simulink model "DLS_ex2"  (R2025b)
settings: Solver=VariableStepAuto  StartTime=0  StopTime=200000  FixedStep=0.5  MaxStep=200  MinStep=0.1  RelTol=.0001
model workspace (MATLAB code in the model file):
  | Temp_Ambient= 295.15;
  | Temp_Environment=295.15;
  | Time_Warmup = 200000;
  | 
  | %material properties: Specific heat and Density
  | Density_Copper = 8960/1000000000;
  | Density_G10 = 1800/1000000000;
  | Density_Stainless_Steel = 7930/1000000000;
  | Density_Aluminium = 2700/1000000000;
  | Density_Titanium = 4500/1000000000;
  | Density_Aluminium_Nitride = 3300/1000000000;
  | Density_Invar = 8050/1000000000;
  | 
  | SHC_Copper = 386;
  | SHC_G10 = 500;
  | SHC_Stainless_Steel = 500;
  | SHC_Aluminium = 900;
  | SHC_Titanium = 528;
  | SHC_Aluminium_Nitride = 820;
  | SHC_Phosphor_Bronze = 377;
  | SHC_Invar = 515;
  | 
  | %Radiation Coefficients
  | K_B1_LB = 2.83489E-08;
  | K_B1_RE = 1.13396E-08;
  | K_B1_UB = 5.66944E-09;
  | 
  | K_B2_LB = 5.15455E-10;
  | K_B2_RE = 2.3625E-10;
  | K_B2_UB = 9.61017E-11;
  | 
  | K_B3_LB = 5.15455E-09;
  | K_B3_RE = 2.3625E-09;
  | K_B3_UB = 9.61017E-10;
  | 
  | K_B4_LB = 5.15455E-09;
  | K_B4_RE = 2.3625E-09;
  | K_B4_UB = 9.61017E-10;
  | 
  | K_B5_LB = 5.15455E-09;
  | K_B5_RE = 2.3625E-09;
  | K_B5_UB = 9.61017E-10;
  | 
  | K_B6_LB = 5.15455E-09;
  | K_B6_RE = 2.3625E-09;
  | K_B6_UB = 9.61017E-10;
  | 
  | K_B7_LB = 5.67E-09;
  | K_B7_RE = 2.8E-09;
  | K_B7_UB = 1.11176E-09;
  | 
  | K_B8_LB = 5.67E-09;
  | K_B8_RE = 2.8E-09;
  | K_B8_UB = 1.11176E-09;
  | 
  | K_B9_LB = 2.835E-08;
  | K_B9_RE = 1.08E-08;
  | K_B9_UB = 5.15455E-09;
  | 
  | K_B10_LB = 4.78193E-09;
  | K_B10_RE = 8.95937E-10;
  | K_B10_UB = 2.20909E-09;
  | 
  | 
  | 
  | 
  | 
  | 
  | 
  | 
  | 
  | K_B13_LB = 3.54375E-09;
  | K_B13_RE = 1.73571E-09;
  | K_B13_UB = 6.85887E-10;
  | 
  | K_B14_LB = 2.98421E-09;
  | K_B14_RE = 1.45385E-09;
  | K_B14_UB = 5.72727E-10;
  | 
  | K_B15_LB = 4.05E-10;
  | K_B15_RE = 1.95517E-10;
  | K_B15_UB = 5.72727E-11;
  | 
  | K_B16_LB = 4.05E-09;
  | K_B16_RE = 1.95517E-09;
  | K_B16_UB = 5.72727E-10;
  | 
  | K_B17_LB = 2.83458E-09;
  | K_B17_RE = 1.13386E-09;
  | K_B17_UB = 5.66908E-10;
  | 
  | K_B18_LB = 2.83458E-09;
  | K_B18_RE = 1.13386E-09;
  | K_B18_UB = 5.66908E-10;
  | 
  | K_B19_LB = 2.83458E-09;
  | K_B19_RE = 1.13386E-09;
  | K_B19_UB = 5.66908E-10;
  | 
  | K_B20_LB = 5.15455E-10;
  | K_B20_RE = 2.3625E-10;
  | K_B20_UB = 9.61017E-11;
  | 
  | K_B21_LB = 9.45E-09;
  | K_B21_RE = 4.05E-09;
  | K_B21_UB = 9.61017E-10;
  | 
  | K_B22_LB = 4.78193E-09;
  | K_B22_RE = 2.20909E-09;
  | K_B22_UB = 8.95937E-10;
  | 
  | K_B23_LB = 5.15455E-09;
  | K_B23_RE = 2.3625E-09;
  | K_B23_UB = 9.61017E-10;
  | 
  | 
  | 
  | 
  | 
  | K_B25_LB = 2.98421E-09;
  | K_B25_RE = 1.45385E-09;
  | K_B25_UB = 5.72727E-10;
  | 
  | K_B1 = K_B1_RE;
  | K_B2 = K_B2_RE;
  | K_B3 = K_B3_RE;
  | K_B4 = K_B4_RE;
  | K_B5 = K_B5_RE;
  | K_B6 = K_B6_RE;
  | K_B7 = K_B7_RE;
  | K_B8 = K_B8_RE;
  | K_B9 = K_B9_RE;
  | K_B10 = K_B10_RE;
  | 
  | 
  | K_B13 = K_B13_RE;
  | K_B14 = K_B14_RE;
  | K_B15 = K_B15_RE;
  | K_B16 = K_B16_RE;
  | K_B17 = K_B17_RE;
  | K_B18 = K_B18_RE;
  | K_B19 = K_B19_RE;
  | K_B20 = K_B20_RE;
  | K_B21 = K_B21_RE;
  | K_B22 = K_B22_RE;
  | K_B23 = K_B23_RE;
  | 
  | K_B25 = K_B25_RE;
  | 
  | %Radiation Surface Area
  | Area_B1 = 100000; %measured 24400 on crude model
  | Area_B2 = 30000; %was 50900
  | Area_B3 = 450;
  | Area_B4 = 613;
  | Area_B5 = 4410;
  | Area_B6 = 1590;
  | Area_B7 = 120;
  | Area_B8 = 50;
  | Area_B9 = 140;
  | Area_B10 = 100;
  | 
  | 
  | Area_B13 = 9990;
  | Area_B14 = 7710;
  | Area_B15 = 10000; %measured 8400 on crude model for 15 and 16 combined
  | Area_B16 = 2000;
  | Area_B17 = 70015;
  | Area_B18 = 16000; %no block model in CAD, estimated value
  | Area_B19 = 320000;
  | Area_B20 = 70000;
  | Area_B21 = 4000; %no CAD, estimated value
  | Area_B22 = 4900;
  | Area_B23 = 9155;
  | 
  | Area_B25 = 4072;
  | 
  | %Akima approximation to calculate contact resistance or fixed resistance values where appropriate
  | xt=linspace(5,295,2000);
  | x_restemp=[4	10	20	30	40	50	60	70	80	90	100	110	120	130	140	150	160	170	180	190	200	210	220	230	240	250	260	273	280	293	300];
  | 
  | y_res_A1_LB=[1.852847068	0.77281194	0.49125288	0.555353451	0.801331659	1.184325573	1.60557094	1.971748902	2.248473254	2.443766462	2.578413714	2.67150152	2.736985932	2.784247759	2.819401592	2.846406384	2.867837824	2.885389229	2.900188421	2.912997223	2.924337653	2.934572526	2.943957542	2.95267538	2.960858317	2.96860341	2.975982825	2.985117154	2.989849299	2.998335893	3.002758516];
  | res_A1_LB=(akima(x_restemp,y_res_A1_LB,xt))';
  | y_res_A1_RE=[1.558179157	0.649907636	0.413126378	0.467032702	0.673891715	0.995976115	1.350228639	1.658171414	1.890886853	2.055121565	2.168355165	2.246638732	2.301708818	2.34145435	2.371017486	2.393727565	2.411750652	2.426510766	2.438956365	2.449728117	2.459265019	2.467872188	2.475764655	2.48309605	2.489977612	2.496490963	2.502696791	2.51037844	2.514358008	2.521494934	2.525214205];
  | res_A1_RE=(akima(x_restemp,y_res_A1_RE,xt))';
  | y_res_A1_UB=[1.383495056	0.577047894	0.366811672	0.414674674	0.59834317	0.884319383	1.198857421	1.472277397	1.67890361	1.824726324	1.925265549	1.994772914	2.043669212	2.078958958	2.105207835	2.125371936	2.141374494	2.154479883	2.165530233	2.175094387	2.183562128	2.191204365	2.198212025	2.204721514	2.210831598	2.216614751	2.222124857	2.228945334	2.23247876	2.238815581	2.242117892];
  | res_A1_UB=(akima(x_restemp,y_res_A1_UB,xt))';
  | 
  | y_res_A2_LB=[0.466691844	0.194654505	0.123735907	0.139881445	0.201838001	0.298305832	0.40440837	0.496640627	0.566341468	0.615531576	0.649446288	0.67289308	0.689387178	0.701291403	0.710145888	0.716947808	0.722345921	0.726766738	0.730494332	0.73372059	0.736576998	0.73915494	0.741518821	0.743714655	0.745775758	0.747726578	0.749585292	0.751886031	0.753077956	0.755215544	0.756329506];
  | res_A2_LB=(akima(x_restemp,y_res_A2_LB,xt))';
  | y_res_A2_RE=[0.422241188	0.17611439	0.111950524	0.12655826	0.182613685	0.269893315	0.365889982	0.449337462	0.512399558	0.556904491	0.587588954	0.608802526	0.623725623	0.634496015	0.642507144	0.648661206	0.653545169	0.657544919	0.660917474	0.663836444	0.666420789	0.668753191	0.670891922	0.67287861	0.674743402	0.676508414	0.678190092	0.680271694	0.681350092	0.683284083	0.684291945];
  | res_A2_RE=(akima(x_restemp,y_res_A2_RE,xt))';
  | y_res_A2_UB=[0.385689258	0.160868789	0.102259362	0.115602558	0.166805463	0.246529603	0.334216178	0.410439904	0.468042936	0.508695235	0.536723452	0.55610064	0.569731897	0.579569934	0.586887568	0.592508894	0.59697007	0.600623576	0.603704181	0.606370465	0.608731093	0.610861588	0.612815176	0.614629884	0.616333247	0.617945468	0.619481569	0.621382974	0.622368019	0.624134591	0.625055206];
  | res_A2_UB=(akima(x_restemp,y_res_A2_UB,xt))';
  | 
  | y_res_A3_LB=[0.466691844	0.194654505	0.123735907	0.139881445	0.201838001	0.298305832	0.40440837	0.496640627	0.566341468	0.615531576	0.649446288	0.67289308	0.689387178	0.701291403	0.710145888	0.716947808	0.722345921	0.726766738	0.730494332	0.73372059	0.736576998	0.73915494	0.741518821	0.743714655	0.745775758	0.747726578	0.749585292	0.751886031	0.753077956	0.755215544	0.756329506];
  | res_A3_LB=(akima(x_restemp,y_res_A3_LB,xt))';
  | y_res_A3_RE=[0.422241188	0.17611439	0.111950524	0.12655826	0.182613685	0.269893315	0.365889982	0.449337462	0.512399558	0.556904491	0.587588954	0.608802526	0.623725623	0.634496015	0.642507144	0.648661206	0.653545169	0.657544919	0.660917474	0.663836444	0.666420789	0.668753191	0.670891922	0.67287861	0.674743402	0.676508414	0.678190092	0.680271694	0.681350092	0.683284083	0.684291945];
  | res_A3_RE=(akima(x_restemp,y_res_A3_RE,xt))';
  | y_res_A3_UB=[0.385689258	0.160868789	0.102259362	0.115602558	0.166805463	0.246529603	0.334216178	0.410439904	0.468042936	0.508695235	0.536723452	0.55610064	0.569731897	0.579569934	0.586887568	0.592508894	0.59697007	0.600623576	0.603704181	0.606370465	0.608731093	0.610861588	0.612815176	0.614629884	0.616333247	0.617945468	0.619481569	0.621382974	0.622368019	0.624134591	0.625055206];
  | res_A3_UB=(akima(x_restemp,y_res_A3_UB,xt))';
  | 
  | y_res_A4_LB=[1.668225823	0.695807472	0.442303498	0.500016965	0.721485431	1.066317096	1.445588764	1.77528005	2.024431055	2.200264872	2.321495613	2.405307971	2.464267391	2.506819958	2.538470996	2.562784978	2.582080948	2.597883497	2.611208069	2.622740577	2.632951025	2.642166076	2.650615951	2.658465127	2.665832701	2.672806057	2.679450173	2.68767434	2.691934966	2.699575939	2.703557883];
  | res_A4_LB=(akima(x_restemp,y_res_A4_LB,xt))';
  | y_res_A4_RE=[1.40291919	0.585149589	0.371961671	0.420496665	0.606743849	0.896735139	1.215689261	1.492948026	1.70247525	1.8503453	1.952296086	2.022779328	2.072362125	2.108147336	2.134764744	2.155211947	2.171439179	2.184728567	2.195934063	2.205632496	2.214219123	2.221968657	2.229074704	2.235675585	2.241871455	2.247735802	2.253323269	2.260239505	2.263822541	2.27024833	2.273597005];
  | res_A4_RE=(akima(x_restemp,y_res_A4_RE,xt))';
  | y_res_A4_UB=[1.245640948	0.519549732	0.330261851	0.373355692	0.538723106	0.796204099	1.079400963	1.325576846	1.511614426	1.642907084	1.733428387	1.796009905	1.840034081	1.87180749	1.895440878	1.913595789	1.928003821	1.939803364	1.949752636	1.958363799	1.965987798	1.972868548	1.979177952	1.985038822	1.990540086	1.995746994	2.000708063	2.006848934	2.010030283	2.015735691	2.018708954];
  | res_A4_UB=(akima(x_restemp,y_res_A4_UB,xt))';
  | 
  | y_res_A5_LB=[1.101209878	0.459308357	0.291968254	0.330065398	0.476258593	0.703884871	0.954245285	1.171877272	1.336343943	1.452413323	1.532438753	1.587763994	1.626683603	1.65477291	1.675666025	1.691715889	1.704453321	1.714884717	1.723680379	1.731293084	1.738033087	1.744116019	1.749693853	1.75487516	1.759738557	1.764341728	1.768727565	1.774156407	1.776968881	1.782012752	1.784641267];
  | res_A5_LB=(akima(x_restemp,y_res_A5_LB,xt))';
  | y_res_A5_RE=[0.951197386	0.396739002	0.252194832	0.285102187	0.41138019	0.607998042	0.824253069	1.012238103	1.154300276	1.254558086	1.323682039	1.37147059	1.405088369	1.429351206	1.447398153	1.461261622	1.472263895	1.481274272	1.488871744	1.495447407	1.501269252	1.506523536	1.511341528	1.515817011	1.520017891	1.523993994	1.527782369	1.532471667	1.534901011	1.53925778	1.541528225];
  | res_A5_RE=(akima(x_restemp,y_res_A5_RE,xt))';
  | y_res_A5_UB=[0.837873198	0.34947213	0.222148729	0.251135552	0.36236899	0.535562094	0.726052831	0.891641619	1.016778724	1.105091973	1.165980605	1.208075702	1.23768831	1.25906051	1.274957372	1.287169169	1.296860648	1.304797543	1.311489863	1.317282112	1.322410351	1.327038648	1.331282632	1.335224913	1.338925306	1.342427703	1.345764737	1.349895359	1.352035275	1.355872985	1.357872932];
  | res_A5_UB=(akima(x_restemp,y_res_A5_UB,xt))';
  | 
  | y_res_A6_LB=[0.466691844	0.194654505	0.123735907	0.139881445	0.201838001	0.298305832	0.40440837	0.496640627	0.566341468	0.615531576	0.649446288	0.67289308	0.689387178	0.701291403	0.710145888	0.716947808	0.722345921	0.726766738	0.730494332	0.73372059	0.736576998	0.73915494	0.741518821	0.743714655	0.745775758	0.747726578	0.749585292	0.751886031	0.753077956	0.755215544	0.756329506];
  | res_A6_LB=(akima(x_restemp,y_res_A6_LB,xt))';
  | y_res_A6_RE=[0.422241188	0.17611439	0.111950524	0.12655826	0.182613685	0.269893315	0.365889982	0.449337462	0.512399558	0.556904491	0.587588954	0.608802526	0.623725623	0.634496015	0.642507144	0.648661206	0.653545169	0.657544919	0.660917474	0.663836444	0.666420789	0.668753191	0.670891922	0.67287861	0.674743402	0.676508414	0.678190092	0.680271694	0.681350092	0.683284083	0.684291945];
  | res_A6_RE=(akima(x_restemp,y_res_A6_RE,xt))';
  | y_res_A6_UB=[0.385689258	0.160868789	0.102259362	0.115602558	0.166805463	0.246529603	0.334216178	0.410439904	0.468042936	0.508695235	0.536723452	0.55610064	0.569731897	0.579569934	0.586887568	0.592508894	0.59697007	0.600623576	0.603704181	0.606370465	0.608731093	0.610861588	0.612815176	0.614629884	0.616333247	0.617945468	0.619481569	0.621382974	0.622368019	0.624134591	0.625055206];
  | res_A6_UB=(akima(x_restemp,y_res_A6_UB,xt))';
  | 
  | y_res_A7_LB=[0.466691844	0.194654505	0.123735907	0.139881445	0.201838001	0.298305832	0.40440837	0.496640627	0.566341468	0.615531576	0.649446288	0.67289308	0.689387178	0.701291403	0.710145888	0.716947808	0.722345921	0.726766738	0.730494332	0.73372059	0.736576998	0.73915494	0.741518821	0.743714655	0.745775758	0.747726578	0.749585292	0.751886031	0.753077956	0.755215544	0.756329506];
  | res_A7_LB=(akima(x_restemp,y_res_A7_LB,xt))';
  | y_res_A7_RE=[0.422241188	0.17611439	0.111950524	0.12655826	0.182613685	0.269893315	0.365889982	0.449337462	0.512399558	0.556904491	0.587588954	0.608802526	0.623725623	0.634496015	0.642507144	0.648661206	0.653545169	0.657544919	0.660917474	0.663836444	0.666420789	0.668753191	0.670891922	0.67287861	0.674743402	0.676508414	0.678190092	0.680271694	0.681350092	0.683284083	0.684291945];
  | res_A7_RE=(akima(x_restemp,y_res_A7_RE,xt))';
  | y_res_A7_UB=[0.385689258	0.160868789	0.102259362	0.115602558	0.166805463	0.246529603	0.334216178	0.410439904	0.468042936	0.508695235	0.536723452	0.55610064	0.569731897	0.579569934	0.586887568	0.592508894	0.59697007	0.600623576	0.603704181	0.606370465	0.608731093	0.610861588	0.612815176	0.614629884	0.616333247	0.617945468	0.619481569	0.621382974	0.622368019	0.624134591	0.625055206];
  | res_A7_UB=(akima(x_restemp,y_res_A7_UB,xt))';
  | 
  | y_res_A8_LB=[2.570275206	1.072047123	0.68146752	0.770388031	1.111609765	1.642900113	2.227252994	2.735216199	3.11908908	3.390000424	3.576783511	3.705915203	3.796755384	3.862317137	3.911082643	3.948543774	3.978273534	4.002620898	4.023150383	4.040918792	4.056650273	4.070848121	4.083867043	4.095960456	4.107311852	4.118055868	4.128292615	4.140963786	4.147528232	4.159300861	4.165435938];
  | res_A8_LB=(akima(x_restemp,y_res_A8_LB,xt))';
  | y_res_A8_RE=[2.177935172	0.908404333	0.577444811	0.652792038	0.941927931	1.392119386	1.887273636	2.317698724	2.642975273	2.872533315	3.030804871	3.140225237	3.217199105	3.272753174	3.314074863	3.345817734	3.371009391	3.391640247	3.409036006	3.424092154	3.437422301	3.449452916	3.460484563	3.470731975	3.480350635	3.48945463	3.498128787	3.508865765	3.514428181	3.524403775	3.529602362];
  | res_A8_RE=(akima(x_restemp,y_res_A8_RE,xt))';
  | y_res_A8_UB=[1.891515301	0.788940239	0.501505146	0.566943472	0.818055154	1.20904201	1.639078612	2.012898573	2.29539806	2.494766965	2.632224255	2.727254769	2.794105817	2.84235398	2.878241461	2.905809833	2.927688539	2.945606235	2.960714281	2.973790398	2.985367499	2.99581597	3.005396847	3.014296624	3.022650336	3.030557066	3.038090486	3.047415446	3.052246349	3.060910055	3.065424976];
  | res_A8_UB=(akima(x_restemp,y_res_A8_UB,xt))';
  | 
  | y_res_A9_LB=[1.302482525	0.543258029	0.34533249	0.390392805	0.56330633	0.832536797	1.128656611	1.386066089	1.580593009	1.717876865	1.812528872	1.877966134	1.923999239	1.957222544	1.98193438	2.000917743	2.015983248	2.028321232	2.038724514	2.047728624	2.055700525	2.06289526	2.069492577	2.075620893	2.081373193	2.086817704	2.092005158	2.098426252	2.101752774	2.107718533	2.110827473];
  | res_A9_LB=(akima(x_restemp,y_res_A9_LB,xt))';
  | y_res_A9_RE=[1.095341951	0.456860878	0.290412467	0.328306606	0.473720793	0.700134138	0.949160477	1.165632786	1.329223078	1.444673968	1.524272974	1.579303408	1.618015628	1.645955258	1.666737042	1.682701383	1.695370942	1.705746752	1.714495546	1.722067686	1.728771774	1.734822293	1.740370404	1.745524102	1.750361583	1.754940226	1.759302692	1.764702606	1.767500094	1.772517088	1.775131596];
  | res_A9_RE=(akima(x_restemp,y_res_A9_RE,xt))';
  | y_res_A9_UB=[0.946128819	0.394624932	0.250850982	0.283582986	0.409188103	0.604758253	0.819860939	1.006844274	1.148149452	1.247873026	1.316628644	1.364162548	1.397601191	1.42173474	1.439685522	1.453475118	1.464418764	1.473381128	1.480938116	1.48747874	1.493269562	1.498495848	1.503288167	1.507739802	1.511918297	1.515873213	1.519641402	1.524305712	1.526722111	1.531055664	1.533314011];
  | res_A9_UB=(akima(x_restemp,y_res_A9_UB,xt))';
  | 
  | y_res_A10_LB=[21.77846125	8.966644519	5.100967849	4.830535038	5.997610209	8.079798747	10.41365885	12.43492555	13.94699339	15.00095825	15.71759461	16.20529908	16.54225342	16.78052084	16.95380548	17.08380935	17.18458127	17.26531026	17.33208171	17.38897845	17.43877523	17.48338116	17.52412521	17.56194268	17.59749867	17.63127075	17.6636051	17.69475498	17.72490735	17.75420153	17.78274238];
  | res_A10_LB=(akima(x_restemp,y_res_A10_LB,xt))';
  | y_res_A10_RE=[19.70414413	8.112605106	4.615119706	4.370444611	5.426360229	7.310228083	9.421796722	11.25054532	12.61859435	13.57217298	14.2205524	14.66180485	14.96666555	15.18223888	15.33901881	15.45664029	15.54781407	15.62085392	15.68126564	15.73274318	15.777797	15.81815438	15.85501771	15.88923321	15.92140262	15.95195804	15.98121267	16.00939564	16.03667611	16.06318013	16.08900256];
  | res_A10_RE=(akima(x_restemp,y_res_A10_RE,xt))';
  | y_res_A10_UB=[17.99842591	7.410325513	4.215605081	3.992110645	4.956619375	6.677407437	8.606185031	10.27662531	11.52624717	12.39727787	12.98952937	13.39258415	13.67105413	13.86796604	14.01117409	14.11861349	14.20189467	14.26861172	14.32379381	14.37081513	14.4119688	14.44883258	14.48250478	14.51375837	14.54314299	14.57105333	14.59777549	14.62351876	14.64843765	14.67264731	14.69623439];
  | res_A10_UB=(akima(x_restemp,y_res_A10_UB,xt))';
  | 
  | res_A11_LB = 1;
  | res_A11_RE = 1;
  | res_A11_UB = 1;
  | 
  | y_res_A12_LB=[0.342532347	0.142868287	0.090816994	0.102667146	0.148140674	0.218944038	0.296818875	0.364513505	0.415671015	0.451774502	0.476666486	0.493875453	0.505981433	0.514718638	0.521217461	0.526209786	0.530171776	0.533416471	0.53615237	0.538520309	0.540616793	0.542508894	0.544243885	0.545855535	0.547368299	0.54880012	0.550164338	0.551852985	0.552727807	0.554296708	0.55511431];
  | res_A12_LB=(akima(x_restemp,y_res_A12_LB,xt))';
  | y_res_A12_RE=[0.342532347	0.142868287	0.090816994	0.102667146	0.148140674	0.218944038	0.296818875	0.364513505	0.415671015	0.451774502	0.476666486	0.493875453	0.505981433	0.514718638	0.521217461	0.526209786	0.530171776	0.533416471	0.53615237	0.538520309	0.540616793	0.542508894	0.544243885	0.545855535	0.547368299	0.54880012	0.550164338	0.551852985	0.552727807	0.554296708	0.55511431];
  | res_A12_RE=(akima(x_restemp,y_res_A12_RE,xt))';
  | y_res_A12_UB=[0.342532347	0.142868287	0.090816994	0.102667146	0.148140674	0.218944038	0.296818875	0.364513505	0.415671015	0.451774502	0.476666486	0.493875453	0.505981433	0.514718638	0.521217461	0.526209786	0.530171776	0.533416471	0.53615237	0.538520309	0.540616793	0.542508894	0.544243885	0.545855535	0.547368299	0.54880012	0.550164338	0.551852985	0.552727807	0.554296708	0.55511431];
  | res_A12_UB=(akima(x_restemp,y_res_A12_UB,xt))';
  | 
  | res_A13_LB = 7238;
  | res_A13_RE = 10000;
  | res_A13_UB = 30000;
  | 
  | y_res_A14_LB=[3232.518226	329.2505618	95.9646967	56.16367989	39.40139945	30.08010454	24.15548607	20.07156297	17.09584808	14.83878298	13.07413448	11.66127195	10.50803612	9.55148427	8.747184396	8.062910655	7.474752995	6.964623057	6.518603596	6.125826366	5.777691393	5.467312659	5.189117438	4.938552014	4.711862405	4.505928832	4.318139263	4.14629174	3.988518194	3.843224457	3.709042615];
  | res_A14_LB=(akima(x_restemp,y_res_A14_LB,xt))';
  | y_res_A14_RE=[6244.813576	636.0701578	185.3915737	108.5010775	76.11848627	58.1109315	46.66532307	38.7757037	33.02700148	28.66663912	25.25756293	22.52809243	20.30018767	18.4522513	16.89844637	15.57651664	14.44027093	13.45476486	12.59311205	11.83431646	11.16176403	10.56215184	10.0247141	9.540653605	9.102718147	8.70488071	8.342095175	8.010107643	7.705309245	7.424620246	7.165398014];
  | res_A14_RE=(akima(x_restemp,y_res_A14_RE,xt))';
  | y_res_A14_UB=[55656.95959	5668.981249	1652.30414	967.0168715	678.406723	517.9142221	415.9051296	345.588823	294.3534605	255.4916901	225.1082666	200.7818351	180.9256131	164.4558628	150.6075618	138.8258506	128.6990502	119.915718	112.2362293	105.4734565	99.47932661	94.13527734	89.34535844	85.03116475	81.12806088	77.58233099	74.34900151	71.39015952	68.67364093	66.17199759	63.86167702];
  | res_A14_UB=(akima(x_restemp,y_res_A14_UB,xt))';
  | 
  | y_res_A15_LB=[18852.89253	1919.826452	559.4350096	327.3742072	229.6417167	175.2952947	140.7570266	116.9536284	99.61203319	86.45950823	76.17664631	67.94366255	61.22351011	55.64945847	50.96263823	46.97528904	43.54809249	40.57564411	37.97683973	35.68833978	33.66002165	31.85175061	30.23104551	28.77136414	27.4508255	26.25124518	25.1573983	24.15808684	23.237513	22.39281994	21.6098224];
  | res_A15_LB=(akima(x_restemp,y_res_A15_LB,xt))';
  | y_res_A15_RE=[36421.38759	3708.86023	1080.757199	632.4452798	443.6385535	338.6481869	271.9246512	225.9395169	192.4377633	167.02876	147.1635802	131.2585039	118.2760252	107.5076672	98.45332737	90.7502765	84.12936919	78.38697743	73.36641831	68.94532783	65.0268755	61.53352611	58.40253024	55.5826117	53.03149923	50.7140628	48.60088992	46.67034743	44.891916	43.26007657	41.74742503];
  | res_A15_RE=(akima(x_restemp,y_res_A15_RE,xt))';
  | y_res_A15_UB=[86976.01305	8856.935365	2580.899808	1510.309534	1059.430054	808.7080442	649.3690541	539.5543571	459.5505696	398.872656	351.433658	313.4515763	282.448797	256.7334439	235.1112479	216.7159945	200.9049516	187.1918459	175.2025109	164.6447357	155.2872844	146.9449992	139.4680315	132.7339314	126.6417529	121.1076041	116.0612463	111.4510186	107.2040394	103.307129	99.69484483];
  | res_A15_UB=(akima(x_restemp,y_res_A15_UB,xt))';
  | 
  | res_A16_LB = 3200;
  | res_A16_RE = 15000;
  | res_A16_UB = 100000;
  | 
  | res_A17_LB = 113.53;
  | res_A17_RE = 135;
  | res_A17_UB = 166.88;
  | 
  | res_A18_LB = 113.16;
  | res_A18_RE = 134.55;
  | res_A18_UB = 166.33;
  | 
  | res_A19_LB = 2611.7;
  | res_A19_RE = 2974.3;
  | res_A19_UB = 3458;
  | 
  | y_res_A20_LB=[3.730185699	1.555839171	0.988999307	1.118047753	1.613255593	2.384305966	3.232364864	3.969561053	4.526667594	4.919835462	5.19090978	5.378315857	5.510150278	5.605298654	5.676070995	5.730437537	5.773583705	5.808918516	5.838712521	5.864499435	5.887330198	5.907935233	5.926829318	5.94438023	5.960854269	5.976446831	5.991303204	6.009692605	6.019219446	6.036304812	6.045208518];
  | res_A20_LB=(akima(x_restemp,y_res_A20_LB,xt))';
  | y_res_A20_RE=[3.136954858	1.308405972	0.831713601	0.940238801	1.356691161	2.005117381	2.71830506	3.338261103	3.806768092	4.137408428	4.365372387	4.5229743	4.633842407	4.713858842	4.77337589	4.819096238	4.855380646	4.885095978	4.910151687	4.931837574	4.951037442	4.968365551	4.984254811	4.999014511	5.012868597	5.025981393	5.03847508	5.053939918	5.061951657	5.076319848	5.083807551];
  | res_A20_RE=(akima(x_restemp,y_res_A20_RE,xt))';
  | y_res_A20_UB=[2.785277622	1.161723404	0.738471985	0.834830659	1.204595444	1.780328001	2.413561749	2.964015859	3.379999541	3.673572502	3.875979914	4.015913417	4.11435234	4.185398305	4.238243025	4.278837763	4.311054405	4.337438415	4.359685183	4.378939912	4.395987324	4.411372816	4.425480766	4.438585787	4.450886722	4.462529471	4.473622518	4.487353626	4.494467186	4.50722459	4.513872863];
  | res_A20_UB=(akima(x_restemp,y_res_A20_UB,xt))';
  | 
  | y_res_A21_LB=[5.996914074	2.501278643	1.589986221	1.797453759	2.5935854	3.833181282	5.196581594	6.381751062	7.277395496	7.909480359	8.345278875	8.646566326	8.858512797	9.01148015	9.125258843	9.212662395	9.282027269	9.338834045	9.386733025	9.428189918	9.464894289	9.498020421	9.528395908	9.556612013	9.583096859	9.608164581	9.632048752	9.661612871	9.676928904	9.704396563	9.7187108];
  | res_A21_LB=(akima(x_restemp,y_res_A21_LB,xt))';
  | y_res_A21_RE=[3.802468989	1.585988119	1.00816407	1.139713208	1.644517152	2.430508888	3.295001415	4.046482942	4.614385057	5.015171705	5.291498884	5.482536503	5.616925602	5.713917757	5.78606152	5.841481574	5.885463825	5.921483351	5.951854703	5.978141314	6.001414489	6.022418808	6.041679021	6.059570034	6.076363305	6.09225802	6.107402278	6.126148027	6.135859479	6.153275924	6.162352165];
  | res_A21_RE=(akima(x_restemp,y_res_A21_RE,xt))';
  | y_res_A21_UB=[3.349448705	1.397035944	0.888052959	1.003929536	1.448591918	2.140941812	2.902440034	3.564391213	4.064634347	4.417671892	4.661077877	4.82935557	4.947733759	5.033170419	5.096719085	5.145536479	5.184278753	5.216006969	5.242759924	5.265914789	5.286415234	5.30491713	5.321882712	5.337642217	5.352434764	5.366435807	5.379775802	5.396288211	5.404842655	5.420184132	5.428179044];
  | res_A21_UB=(akima(x_restemp,y_res_A21_UB,xt))';
  | 
  | y_res_A22_LB=[0.466691844	0.194654505	0.123735907	0.139881445	0.201838001	0.298305832	0.40440837	0.496640627	0.566341468	0.615531576	0.649446288	0.67289308	0.689387178	0.701291403	0.710145888	0.716947808	0.722345921	0.726766738	0.730494332	0.73372059	0.736576998	0.73915494	0.741518821	0.743714655	0.745775758	0.747726578	0.749585292	0.751886031	0.753077956	0.755215544	0.756329506];
  | res_A22_LB=(akima(x_restemp,y_res_A22_LB,xt))';
  | y_res_A22_RE=[0.422241188	0.17611439	0.111950524	0.12655826	0.182613685	0.269893315	0.365889982	0.449337462	0.512399558	0.556904491	0.587588954	0.608802526	0.623725623	0.634496015	0.642507144	0.648661206	0.653545169	0.657544919	0.660917474	0.663836444	0.666420789	0.668753191	0.670891922	0.67287861	0.674743402	0.676508414	0.678190092	0.680271694	0.681350092	0.683284083	0.684291945];
  | res_A22_RE=(akima(x_restemp,y_res_A22_RE,xt))';
  | y_res_A22_UB=[0.385689258	0.160868789	0.102259362	0.115602558	0.166805463	0.246529603	0.334216178	0.410439904	0.468042936	0.508695235	0.536723452	0.55610064	0.569731897	0.579569934	0.586887568	0.592508894	0.59697007	0.600623576	0.603704181	0.606370465	0.608731093	0.610861588	0.612815176	0.614629884	0.616333247	0.617945468	0.619481569	0.621382974	0.622368019	0.624134591	0.625055206];
  | res_A22_UB=(akima(x_restemp,y_res_A22_UB,xt))';
  | 
  | y_res_A23_LB=[0.466691844	0.194654505	0.123735907	0.139881445	0.201838001	0.298305832	0.40440837	0.496640627	0.566341468	0.615531576	0.649446288	0.67289308	0.689387178	0.701291403	0.710145888	0.716947808	0.722345921	0.726766738	0.730494332	0.73372059	0.736576998	0.73915494	0.741518821	0.743714655	0.745775758	0.747726578	0.749585292	0.751886031	0.753077956	0.755215544	0.756329506];
  | res_A23_LB=(akima(x_restemp,y_res_A23_LB,xt))';
  | y_res_A23_RE=[0.422241188	0.17611439	0.111950524	0.12655826	0.182613685	0.269893315	0.365889982	0.449337462	0.512399558	0.556904491	0.587588954	0.608802526	0.623725623	0.634496015	0.642507144	0.648661206	0.653545169	0.657544919	0.660917474	0.663836444	0.666420789	0.668753191	0.670891922	0.67287861	0.674743402	0.676508414	0.678190092	0.680271694	0.681350092	0.683284083	0.684291945];
  | res_A23_RE=(akima(x_restemp,y_res_A23_RE,xt))';
  | y_res_A23_UB=[0.385689258	0.160868789	0.102259362	0.115602558	0.166805463	0.246529603	0.334216178	0.410439904	0.468042936	0.508695235	0.536723452	0.55610064	0.569731897	0.579569934	0.586887568	0.592508894	0.59697007	0.600623576	0.603704181	0.606370465	0.608731093	0.610861588	0.612815176	0.614629884	0.616333247	0.617945468	0.619481569	0.621382974	0.622368019	0.624134591	0.625055206];
  | res_A23_UB=(akima(x_restemp,y_res_A23_UB,xt))';
  | 
  | y_res_A24_LB=[5.996914074	2.501278643	1.589986221	1.797453759	2.5935854	3.833181282	5.196581594	6.381751062	7.277395496	7.909480359	8.345278875	8.646566326	8.858512797	9.01148015	9.125258843	9.212662395	9.282027269	9.338834045	9.386733025	9.428189918	9.464894289	9.498020421	9.528395908	9.556612013	9.583096859	9.608164581	9.632048752	9.661612871	9.676928904	9.704396563	9.7187108];
  | res_A24_LB=(akima(x_restemp,y_res_A24_LB,xt))';
  | y_res_A24_RE=[3.802468989	1.585988119	1.00816407	1.139713208	1.644517152	2.430508888	3.295001415	4.046482942	4.614385057	5.015171705	5.291498884	5.482536503	5.616925602	5.713917757	5.78606152	5.841481574	5.885463825	5.921483351	5.951854703	5.978141314	6.001414489	6.022418808	6.041679021	6.059570034	6.076363305	6.09225802	6.107402278	6.126148027	6.135859479	6.153275924	6.162352165];
  | res_A24_RE=(akima(x_restemp,y_res_A24_RE,xt))';
  | y_res_A24_UB=[3.349448705	1.397035944	0.888052959	1.003929536	1.448591918	2.140941812	2.902440034	3.564391213	4.064634347	4.417671892	4.661077877	4.82935557	4.947733759	5.033170419	5.096719085	5.145536479	5.184278753	5.216006969	5.242759924	5.265914789	5.286415234	5.30491713	5.321882712	5.337642217	5.352434764	5.366435807	5.379775802	5.396288211	5.404842655	5.420184132	5.428179044];
  | res_A24_UB=(akima(x_restemp,y_res_A24_UB,xt))';
  | 
  | y_res_A25_LB=[3.385783654	1.412191043	0.897686592	1.014820202	1.464306299	2.164166831	2.933925815	3.603057866	4.108727656	4.465594967	4.711641429	4.881744604	5.001406965	5.087770445	5.15200849	5.201355456	5.240518008	5.272590412	5.299633585	5.323039635	5.34376247	5.362465075	5.3796147	5.395545165	5.410498182	5.424651108	5.438135816	5.454827352	5.463474596	5.478982497	5.487064139];
  | res_A25_LB=(akima(x_restemp,y_res_A25_LB,xt))';
  | y_res_A25_RE=[2.91220524	1.214664189	0.772124821	0.872874647	1.259489947	1.861459157	2.523549939	3.09908874	3.534029174	3.840980521	4.052611821	4.198922221	4.301847094	4.376130688	4.431383589	4.473828267	4.50751305	4.535099403	4.558359977	4.578492161	4.596316439	4.612403062	4.627153924	4.640856153	4.653717652	4.665890972	4.677489539	4.691846386	4.699284117	4.712622888	4.719574129];
  | res_A25_RE=(akima(x_restemp,y_res_A25_RE,xt))';
  | y_res_A25_UB=[2.557152629	1.066573771	0.677988278	0.766454804	1.105934426	1.634512263	2.215881721	2.721251514	3.103164526	3.372692728	3.558522191	3.6869946	3.777370995	3.842598021	3.891114554	3.928384427	3.957962401	3.982185459	4.002610131	4.020287823	4.035938986	4.050064347	4.063016801	4.075048471	4.086341912	4.097031075	4.107215558	4.119822035	4.126352967	4.138065491	4.144169244];
  | res_A25_UB=(akima(x_restemp,y_res_A25_UB,xt))';
  | 
  | y_res_A26_LB=[0.466691844	0.194654505	0.123735907	0.139881445	0.201838001	0.298305832	0.40440837	0.496640627	0.566341468	0.615531576	0.649446288	0.67289308	0.689387178	0.701291403	0.710145888	0.716947808	0.722345921	0.726766738	0.730494332	0.73372059	0.736576998	0.73915494	0.741518821	0.743714655	0.745775758	0.747726578	0.749585292	0.751886031	0.753077956	0.755215544	0.756329506];
  | res_A26_LB=(akima(x_restemp,y_res_A26_LB,xt))';
  | y_res_A26_RE=[0.422241188	0.17611439	0.111950524	0.12655826	0.182613685	0.269893315	0.365889982	0.449337462	0.512399558	0.556904491	0.587588954	0.608802526	0.623725623	0.634496015	0.642507144	0.648661206	0.653545169	0.657544919	0.660917474	0.663836444	0.666420789	0.668753191	0.670891922	0.67287861	0.674743402	0.676508414	0.678190092	0.680271694	0.681350092	0.683284083	0.684291945];
  | res_A26_RE=(akima(x_restemp,y_res_A26_RE,xt))';
  | y_res_A26_UB=[0.385689258	0.160868789	0.102259362	0.115602558	0.166805463	0.246529603	0.334216178	0.410439904	0.468042936	0.508695235	0.536723452	0.55610064	0.569731897	0.579569934	0.586887568	0.592508894	0.59697007	0.600623576	0.603704181	0.606370465	0.608731093	0.610861588	0.612815176	0.614629884	0.616333247	0.617945468	0.619481569	0.621382974	0.622368019	0.624134591	0.625055206];
  | res_A26_UB=(akima(x_restemp,y_res_A26_UB,xt))';
  | 
  | y_res_A27_LB=[0.466691844	0.194654505	0.123735907	0.139881445	0.201838001	0.298305832	0.40440837	0.496640627	0.566341468	0.615531576	0.649446288	0.67289308	0.689387178	0.701291403	0.710145888	0.716947808	0.722345921	0.726766738	0.730494332	0.73372059	0.736576998	0.73915494	0.741518821	0.743714655	0.745775758	0.747726578	0.749585292	0.751886031	0.753077956	0.755215544	0.756329506];
  | res_A27_LB=(akima(x_restemp,y_res_A27_LB,xt))';
  | y_res_A27_RE=[0.422241188	0.17611439	0.111950524	0.12655826	0.182613685	0.269893315	0.365889982	0.449337462	0.512399558	0.556904491	0.587588954	0.608802526	0.623725623	0.634496015	0.642507144	0.648661206	0.653545169	0.657544919	0.660917474	0.663836444	0.666420789	0.668753191	0.670891922	0.67287861	0.674743402	0.676508414	0.678190092	0.680271694	0.681350092	0.683284083	0.684291945];
  | res_A27_RE=(akima(x_restemp,y_res_A27_RE,xt))';
  | y_res_A27_UB=[0.385689258	0.160868789	0.102259362	0.115602558	0.166805463	0.246529603	0.334216178	0.410439904	0.468042936	0.508695235	0.536723452	0.55610064	0.569731897	0.579569934	0.586887568	0.592508894	0.59697007	0.600623576	0.603704181	0.606370465	0.608731093	0.610861588	0.612815176	0.614629884	0.616333247	0.617945468	0.619481569	0.621382974	0.622368019	0.624134591	0.625055206];
  | res_A27_UB=(akima(x_restemp,y_res_A27_UB,xt))';
  | 
  | y_res_A28_LB=[3.385783654	1.412191043	0.897686592	1.014820202	1.464306299	2.164166831	2.933925815	3.603057866	4.108727656	4.465594967	4.711641429	4.881744604	5.001406965	5.087770445	5.15200849	5.201355456	5.240518008	5.272590412	5.299633585	5.323039635	5.34376247	5.362465075	5.3796147	5.395545165	5.410498182	5.424651108	5.438135816	5.454827352	5.463474596	5.478982497	5.487064139];
  | res_A28_LB=(akima(x_restemp,y_res_A28_LB,xt))';
  | y_res_A28_RE=[2.91220524	1.214664189	0.772124821	0.872874647	1.259489947	1.861459157	2.523549939	3.09908874	3.534029174	3.840980521	4.052611821	4.198922221	4.301847094	4.376130688	4.431383589	4.473828267	4.50751305	4.535099403	4.558359977	4.578492161	4.596316439	4.612403062	4.627153924	4.640856153	4.653717652	4.665890972	4.677489539	4.691846386	4.699284117	4.712622888	4.719574129];
  | res_A28_RE=(akima(x_restemp,y_res_A28_RE,xt))';
  | y_res_A28_UB=[2.557152629	1.066573771	0.677988278	0.766454804	1.105934426	1.634512263	2.215881721	2.721251514	3.103164526	3.372692728	3.558522191	3.6869946	3.777370995	3.842598021	3.891114554	3.928384427	3.957962401	3.982185459	4.002610131	4.020287823	4.035938986	4.050064347	4.063016801	4.075048471	4.086341912	4.097031075	4.107215558	4.119822035	4.126352967	4.138065491	4.144169244];
  | res_A28_UB=(akima(x_restemp,y_res_A28_UB,xt))';
  | 
  | res_A31_LB = 113.53;
  | res_A31_RE = 135;
  | res_A31_UB = 166.88;
  | 
  | res_A32_LB = 113.53;
  | res_A32_RE = 135;
  | res_A32_UB = 166.88;
  | 
  | res_A33_LB = 113.53;
  | res_A33_RE = 135;
  | res_A33_UB = 166.88;
  | 
  | res_A34_LB = 106.89;
  | res_A34_RE = 127.1;
  | res_A34_UB = 157.12;
  | 
  | res_A36_LB = 100;
  | res_A36_RE = 100;
  | res_A36_UB = 100;
  | 
  | y_res_A37_LB=[559.0264465	277.2362191	143.0749777	104.5075798	87.00904569	78.13471948	71.71197015	67.96291148	65.29305409	62.842993	60.67239457	58.91033361	57.3420793	55.60751686	53.98751593	52.67332244	51.36613692	50.09621037	48.99723247	48.01630621	46.85892867	45.6703913	44.78832759	44.04526831	43.31563014	42.56138686	41.81566865	40.7882804	40.20917218	39.33052889	38.95803316];
  | res_A37_LB=(akima(x_restemp,y_res_A37_LB,xt))';
  | y_res_A37_RE=[647.1900089	320.958896	165.6392048	120.9893771	100.7311647	90.45727643	83.02160102	78.68128165	75.59036344	72.75390539	70.24098382	68.20102979	66.38544749	64.37732876	62.50183893	60.98038516	59.46704457	57.99683904	56.72454231	55.58891505	54.24900852	52.87302799	51.8518548	50.9916083	50.14689955	49.27370523	48.41038047	47.22096373	46.55052488	45.53331153	45.10206983];
  | res_A37_RE=(akima(x_restemp,y_res_A37_RE,xt))';
  | y_res_A37_UB=[769.5803815	381.6555667	196.963304	143.8697286	119.7804773	107.5636897	98.72185062	93.56073165	89.8852886	86.51242679	83.52428557	81.09855499	78.93962716	76.55175226	74.32158777	72.51241124	70.71288218	68.96464546	67.45174417	66.10135796	64.50806116	62.87186837	61.6575807	60.63465262	59.63020065	58.59187618	57.56528771	56.15093988	55.35371406	54.14413507	53.63134107];
  | res_A37_UB=(akima(x_restemp,y_res_A37_UB,xt))';
  | 
  | y_res_A38_LB=[2345.090752	1130.561947	581.6666576	422.6544105	349.8576636	312.0465495	284.8066406	268.4066012	256.6420417	246.1348008	236.9762773	229.5566373	223.0182223	215.9827861	209.4645901	204.153488	198.9254688	193.8820407	189.5114151	185.6109261	181.0822346	176.460892	172.997342	170.0672492	167.2022427	164.2593883	161.3602236	157.4235406	155.1660155	151.8003204	150.3265927];
  | res_A38_LB=(akima(x_restemp,y_res_A38_LB,xt))';
  | y_res_A38_RE=[2714.932924	1308.861864	673.4007875	489.3108607	405.0334038	361.2591326	329.723242	310.736767	297.1168293	284.9525007	274.3495947	265.7598099	258.1902273	250.0452388	242.4990638	236.3503526	230.2978272	224.4590044	219.3990914	214.8834598	209.6405524	204.290382	200.2805986	196.8884035	193.5715593	190.1645899	186.8082006	182.2506669	179.6371095	175.7406136	174.0344656];
  | res_A38_RE=(akima(x_restemp,y_res_A38_RE,xt))';
  | y_res_A38_UB=[3228.355021	1556.381277	800.7478913	581.8446417	481.6294397	429.5769979	392.0773418	369.5003266	353.3047168	338.839987	326.231961	316.0177584	307.0166889	297.3313982	288.358163	281.0466664	273.8495453	266.9065404	260.8897451	255.5201605	249.2857647	242.9238213	238.1557461	234.1220516	230.1779576	226.1266948	222.1355773	216.7161665	213.6083582	208.9749944	206.946196];
  | res_A38_UB=(akima(x_restemp,y_res_A38_UB,xt))';
  | 
  | res_A1 = res_A1_RE;
  | res_A2 = res_A2_RE;
  | res_A3 = res_A3_RE;
  | res_A4 = res_A4_RE;
  | res_A5 = res_A5_RE;
  | res_A6 = res_A6_RE;
  | res_A7 = res_A7_RE;
  | res_A8 = res_A8_RE;
  | res_A9 = res_A9_RE;
  | res_A10 = res_A10_RE;
  | res_A11 = res_A11_RE;
  | res_A12 = res_A12_RE;
  | res_A13 = res_A13_RE;
  | res_A14 = res_A14_RE;
  | res_A15 = res_A15_RE;
  | res_A16 = res_A16_RE;
  | res_A17 = res_A17_RE;
  | res_A18 = res_A18_RE;
  | res_A19 = res_A19_RE;
  | res_A20 = res_A20_RE;
  | res_A21 = res_A21_RE;
  | res_A22 = res_A22_RE;
  | res_A23 = res_A23_RE;
  | res_A24 = res_A24_RE;
  | res_A25 = res_A25_RE;
  | res_A26 = res_A26_RE;
  | res_A27 = res_A27_RE;
  | res_A28 = res_A28_RE;
  | 
  | res_A31 = res_A31_RE;
  | res_A32 = res_A32_RE;
  | res_A33 = res_A33_RE;
  | res_A34 = res_A34_RE;
  | 
  | res_A36 = res_A36_RE;
  | res_A37 = res_A37_RE;
  | res_A38 = res_A38_RE;
  | 
  | %Component Geometry
  | Length_1_2_1 = 35;
  | Length_1_2_2 = 280;
  | Length_1_2_3 = 25.4;
  | Length_1_3 = 442;
  | Length_1_4_1 = 25.4;
  | Length_1_4_2_3D = 370;
  | Length_1_4_2_2D = 100;
  | Length_1_4_2 = Length_1_4_2_2D;
  | Length_1_4_3 = 25.4;
  | Length_1_5_1 = 10.5;
  | Length_1_5_2 = 14;
  | Length_1_6_1 = 2.5;
  | Length_1_6_2 = 4.55;
  | Length_1_6_3 = 2.5;
  | Length_1_7 = 2;
  | Length_1_8 = 0.25;
  | 
  | Length_2_2 = 1.5;
  | Length_2_3_1 = 25;
  | Length_2_3_2 = 285;
  | Length_2_3_3 = 25;
  | Length_2_4_1 = 270;
  | Length_2_4_2 = 390;
  | Length_2_4_3 = 150;
  | Length_2_5_1 = 25;
  | Length_2_5_2 = 50;
  | Length_2_5_3 = 25;
  | Length_2_6 = 25;
  | 
  | Length_3_1 = 10;
  | 
  | %Length_4_1 = 5;
  | Length_4_2 = 5;
  | Length_4_3 = 5;
  | Length_4_4 = 25;
  | Length_4_7_1 = 5.5; %outer ring
  | Length_4_7_2 = 12.3; %outer arm
  | Length_4_7_3 = 36.3; %inner ring arm
  | Length_4_7_4 = 12; %flexure
  | Length_4_7_5 = 1.1; %inner arm
  | Length_4_7_6 = 5.8; %connector
  | 
  | Length_7_1_1 = 170;
  | Length_7_1_2 = 50;
  | Length_7_1_3_1 = 1;
  | Length_7_1_3_2 = 1;
  | Length_7_3 = 12;
  | Length_7_4_1 = 12;
  | Length_7_4_2 = 12;
  | 
  | Area_1_2_1 = 711.2;
  | Area_1_2_2 = 232.6;
  | Area_1_2_3 = 711.2;
  | Area_1_3 = 560;
  | Area_1_4_1 = 160;
  | Area_1_4_2 = 12.9;
  | Area_1_4_3 = 160;
  | Area_1_5_1 = 43.5;
  | Area_1_5_2 = 300;
  | Area_1_6_1 = 291.2;
  | Area_1_6_2 = 1040;
  | Area_1_6_3 = 1040;
  | Area_1_7 = 40;
  | Area_1_8 = 0.62;
  | 
  | Area_2_2 = 39100;
  | Area_2_3_1 = 230;
  | Area_2_3_2 = 230;
  | Area_2_3_3 = 230;
  | Area_2_4_1 = 1230;
  | Area_2_4_2 = 220;
  | Area_2_4_3 = 1000;
  | Area_2_5_1 = 161;
  | Area_2_5_2 = 25;
  | Area_2_5_3 = 161;
  | Area_2_6 = 150;
  | 
  | Area_3_1 = 50;
  | 
  | %Area_4_1 = 1*5;
  | Area_4_2 = 6*5;
  | Area_4_3 = 6*5;
  | Area_4_4 = 6*4;
  | Area_4_7_1 = 650.3;
  | Area_4_7_2 = 6;
  | Area_4_7_3 = 6;
  | Area_4_7_4 = 0.8;
  | Area_4_7_5 = 8;
  | Area_4_7_6 = 30;
  | 
  | 
  | Area_7_1_1 = 0.0544;
  | Area_7_1_2 = 0.0544;
  | Area_7_1_3_1 = 0.0544;
  | Area_7_1_3_2 = 20;
  | Area_7_3 = 33.6;
  | Area_7_4_1 = 33.6;
  | Area_7_4_2 = 33.6;
  | 
  | Mass_1_2_1 = Length_1_2_1*Area_1_2_1*Density_Copper;
  | Mass_1_2_2 = Length_1_2_2*Area_1_2_2*Density_Copper;
  | Mass_1_2_3 = Length_1_2_3*Area_1_2_3*Density_Copper;
  | Mass_1_3 = Length_1_3*Area_1_3*Density_Copper;
  | Mass_1_4_1 = Length_1_4_1*Area_1_4_1*Density_Copper;
  | Mass_1_4_2 = Length_1_4_2*Area_1_4_2*Density_Copper;
  | Mass_1_4_3 = Length_1_4_3*Area_1_4_3*Density_Copper;
  | Mass_1_5_1 = Length_1_5_1*Area_1_5_1*Density_Copper;
  | Mass_1_5_2 = Length_1_5_2*Area_1_5_2*Density_Copper;
  | Mass_1_6_1 = Length_1_6_1*Area_1_6_1*Density_Copper;
  | Mass_1_6_2 = Length_1_6_2*Area_1_6_2*Density_Copper;
  | Mass_1_6_3 = Length_1_6_3*Area_1_6_3*Density_Copper;
  | Mass_1_7 = Length_1_7*Area_1_7*Density_Copper;
  | Mass_1_8 = Length_1_8*Area_1_8*Density_Copper;
  | 
  | Mass_2_2 = Length_2_2*Area_2_2*Density_Copper;
  | Mass_2_3_1 = Length_2_3_1*Area_2_3_1*Density_Copper;
  | Mass_2_3_2 = Length_2_3_2*Area_2_3_2*Density_Copper;
  | Mass_2_3_3 = Length_2_3_3*Area_2_3_3*Density_Copper;
  | Mass_2_4_1 = Length_2_4_1*Area_2_4_1*Density_Copper;
  | Mass_2_4_2 = Length_2_4_2*Area_2_4_2*Density_Copper;
  | Mass_2_4_3 = Length_2_4_3*Area_2_4_3*Density_Copper;
  | Mass_2_5_1 = Length_2_5_1*Area_2_5_1*Density_Copper;
  | Mass_2_5_2 = Length_2_5_2*Area_2_5_2*Density_Copper;
  | Mass_2_5_3 = Length_2_5_3*Area_2_5_3*Density_Copper;
  | Mass_2_6 = Length_2_6*Area_2_6*Density_Copper;
  | 
  | Mass_3_1 = Length_3_1*Area_3_1*Density_Aluminium;
  | 
  | %Mass_4_1 = Length_4_1*Area_4_1*Density_G10;
  | Mass_4_2 = Length_4_2*Area_4_2*Density_G10;
  | Mass_4_3 = Length_4_3*Area_4_3*Density_G10;
  | Mass_4_4 = Length_4_4*Area_4_4*Density_G10;
  | Mass_4_7_1 = Length_4_7_1*Area_4_7_1*Density_Titanium;
  | Mass_4_7_2 = Length_4_7_2*Area_4_7_2*Density_Titanium;
  | Mass_4_7_3 = Length_4_7_3*Area_4_7_3*Density_Titanium;
  | Mass_4_7_4 = Length_4_7_4*Area_4_7_4*Density_Titanium;
  | Mass_4_7_5 = Length_4_7_5*Area_4_7_5*Density_Titanium;
  | Mass_4_7_6 = Length_4_7_6*Area_4_7_6*Density_Titanium;
  | 
  | Mass_4_7 = Mass_4_7_1+(6*Mass_4_7_2)+(3*Mass_4_7_3)+(6*Mass_4_7_4)+(3*Mass_4_7_5)+(3*Mass_4_7_6);
  | 
  | %no phosphor bronze or Polyimide in code (being lazy)
  | Mass_7_1_1 = Length_7_1_1*Area_7_1_1*Density_G10;
  | Mass_7_1_2 = Length_7_1_2*Area_7_1_2*Density_G10;
  | Mass_7_1_3 = Length_7_1_3_2*Area_7_1_3_2*Density_G10;
  | Mass_7_3 = Length_7_3*Area_7_3*Density_Copper;
  | Mass_7_4 = Length_7_4_2*Area_7_4_2*Density_Copper;
  | 
  | %Material Conductivities - Akima
  | x_Copper=[4	10	20	30	40	50	60	70	80	90	100	110	120	130	140	150	160	170	180	190	200	210	220	230	240	250	260	270	280	290	300];
  | y_Copper=[1300	1539.915576	2422.510265	2142.896819	1485.109355	1004.846277	741.2099419	603.5581619	529.2769842	486.9798983	461.5493381	445.4667663	434.8086444	427.4278894	422.0984859	418.093899	414.9694705	412.4452713	410.3406298	408.5363123	406.9520296	405.5327079	404.2399139	403.0463867	401.9324857	400.8838429	399.8897888	398.9422797	398.0351596	397.1636446	396.323959];
  | Cond_Copper=(akima(x_Copper,y_Copper,xt))';
  | x_Stainless_Steel=[4	10	20	30	40	50	60	70	80	90	100	110	120	130	140	150	160	170	180	190	200	210	220	230	240	250	260	270	280	290	300];
  | y_Stainless_Steel=[0.272396189	0.903857571	2.168622406	3.468572587	4.670281	5.730166936	6.646641427	7.434751536	8.114319471	8.704844967	9.223590217	9.685093439	10.10128078	10.48179376	10.83436242	11.16515436	11.4790756	11.78001966	12.07106923	12.35465738	12.63269588	12.90667672	13.17775271	13.44680137	13.7144757	13.98124475	14.24742608	14.51321188	14.77869006	15.04386145	15.30865382];
  | Cond_Stainless_Steel=(akima(x_Stainless_Steel,y_Stainless_Steel,xt))';
  | x_G10=[4	10	20	30	40	50	60	70	80	90	100	110	120	130	140	150	160	170	180	190	200	210	220	230	240	250	260	273	280	290	300];
  | y_G10=[0.072322856	0.112201845	0.15642187	0.191111597	0.217459505	0.238163639	0.255310109	0.270284605	0.283977369	0.296959296	0.309599321	0.32213809	0.334733685	0.347490177	0.36047569	0.373733984	0.387292023	0.401164973	0.415359572	0.429876425	0.444711587	0.459857685	0.475304701	0.491040551	0.507051498	0.523322473	0.539837305	0.561642965	0.573529445	0.590670406	0.607982755];
  | Cond_G10=(akima(x_G10,y_G10,xt))';
  | %x_Titanium=[2.0515	2.2546	2.4392	2.6388	2.8548	3.3943	4.3661	5.5284	6.7832	8.3229	10.212	13.989	17.994	23.512	33.766	52.459	78.976	117.04	181.84	241.37	310.48];
  | %y_Titanium=[0.12232	0.13924	0.1551	0.16909	0.18836	0.23375	0.31623	0.42781	0.51955	0.65879	0.81752	1.1301	1.4643	1.8973	2.5119	3.3982	4.403	5.7049	7.5531	9.1728	10.902];
  | %Cond_Titanium=(akima(x_Titanium,y_Titanium,xt))';
  | x_Ti6Al4V = [3.386124876 20.75387993 27.4220298	36.75105129	43.85874494	52.73850131	64.27774056	76.69884488	88.67346161	105.0768464	120.1449347	132.5535402	150.7206551	168.4454488	181.2949868	194.5896236	208.7702918	225.6104428	238.0176595	250.4276537	268.1524474	283.662857	294.7403323 295];
  | y_Ti6Al4V = [0.205026155 1.358500785 1.684540973	2.078506201	2.377376374	2.703416562	3.083796782	3.437006986	3.749462166	4.116257378	4.401542543	4.632487677	4.944942857	5.257398038	5.474758163	5.719288305	5.977403454	6.289858634	6.50721876	6.751748901	7.064204082	7.349489246	7.539679356 7.543];
  | Cond_Titanium=(akima(x_Ti6Al4V,y_Ti6Al4V,xt))';
  | x_Aluminium=[4	10	20	30	40	50	60	70	80	90	100	110	120	130	140	150	160	170	180	190	200	210	220	230	240	250	260	270	280	290	300];
  | y_Aluminium=[5.347423899	14.20430536	28.42754763	41.098463	52.23304247	62.04805557	70.75945479	78.548489	85.56117329	91.91421797	97.70122297	102.9978192	107.8656678	112.3555088	116.5094768	120.3628668	123.9454888	127.2827167	130.3963069	133.3050423	136.0252443	138.5711815	140.9554008	143.1889946	145.2818209	147.2426834	149.0794814	150.799334	152.4086848	153.9133894	155.3187898];
  | Cond_Aluminium=(akima(x_Aluminium,y_Aluminium,xt))';
  | x_Aluminium_Nitride=[4.510967205	5.519278711	6.893424895	8.194672663	11.02220728	15.96576668	18.06467613	20.95070596	24.90549764	30.3472866	35.19559795	39.98681034	49.94240884	59.61479584	70.28693352	79.85516497	99.32709193	124.5685636	149.9232744	175.3127763	200	225.3628799	247.746023	273.4758701	289.7018044 296];
  | y_Aluminium_Nitride=[0.146286823	0.259224634	0.485333553	0.77895911	1.720179013	4.383096438	5.835067139	8.207464275	11.80186514	17.15921944	22.34846936	28.47245162	39.61964949	50.48375339	60.88500046	68.73555234	83.82675	93.62855647	100.0662615	100.1129163	101.2590518	101.2950791	99.12069462	96.99417489	95.95043888 95];
  | Cond_Aluminium_Nitride=(akima(x_Aluminium_Nitride,y_Aluminium_Nitride,xt))';
  | x_Phosphor_Bronze = [4 10	20	30	40	50	60	70	80	90	100	110	120	130	140	150	160	170	180	190	200	210	220	230	240	250	260	270	280	290 300];
  | y_Phosphor_Bronze = [1 4.393242753	9.479425007	13.56115329	16.94081133	19.93208133	22.70978973	25.3722085	27.97919185	30.57036336	33.17382604	35.81054343	38.49667497	41.24489339	44.06516619	46.96523874	49.95094198	53.02639195	56.19412002	59.45515736	62.80908905	66.25408831	69.78693823	73.40304697	77.09646061	80.85987755	84.68466721	88.5608958	92.47736095	96.42163718	98.3801333];
  | Cond_Phosphor_Bronze=(akima(x_Phosphor_Bronze,y_Phosphor_Bronze,xt))';
  | x_Invar = [4	10	20	30	40	50	60	70	80	90	100	110	120	130	140	150	160	170	180	190	200	210	220	230	240	250	260	270	280	290	300];
  | y_Invar = [0.241863429	0.733851185	1.652068813	2.570059877	3.43704896	4.247347833	5.005323106	5.716516689	6.385642999	7.016349158	7.611390432	8.172859892	8.702383399	9.201266957	9.670602925	10.11134476	10.52435878	10.9104594	11.27043275	11.60505191	11.91508648	12.20130795	12.46449231	12.70542074	12.92487899	13.12365589	13.3025415	13.46232477	13.60379132	13.72772106	13.83488599];
  | Cond_Invar =(akima(x_Invar,y_Invar,xt))';
  | x_ti_15_3_3_3 = [1.425338153	1.621392126	1.820795595	2.031588851	2.23775962	2.545561431	2.877101768	3.33672869	3.820230365	4.345699594	4.84880064	5.480320658	6.15430626	6.778860806	7.661756725	8.54875725	9.295731738	10.30527775	11.57265046	12.74707226	14.13144482	15.66616465	17.36755992	19.25373213	21.07143098	22.91261337	25.40099601	27.97875325	30.81810781	33.94560725	37.15033091	40.65760489	44.78364134	49.01155791	55.03914031	61.01656589	68.08044535	77.94549955	87.53146134	96.41437516	106.1987495	119.2593773	130.5183701	141.9228222	151.3691295	160.4072083	171.0838265	181.2990475	190.8901776	211.6214577	219.9635632	231.6001338	242.2860213	251.8369222	297.7697642];
  | y_ti_15_3_3_3 = [0.028183829	0.036192676	0.045927094	0.055568361	0.062596741	0.070514083	0.077563103	0.086338977	0.094969949	0.108263673	0.119086373	0.130990976	0.145811945	0.1603882	0.180674371	0.201116766	0.216014428	0.240455371	0.267661685	0.294418786	0.323850691	0.360492764	0.396529828	0.436169378	0.474091391	0.515310469	0.573615251	0.638516925	0.702346988	0.772557894	0.83972664	0.934737476	1.04049831	1.144512894	1.289272821	1.45234223	1.616667433	1.842965653	2.027199786	2.203451259	2.366671228	2.66601181	2.897803719	3.075608373	3.264322838	3.423597958	3.633664514	3.81096081	3.949587358	4.242151817	4.556387898	4.722129913	4.952535374	5.011872336	5.992198712];
  | Cond_ti_15_3_3_3 =(akima(x_ti_15_3_3_3,y_ti_15_3_3_3,xt))';
  | x_Inconel_718 = [1.993355482	5.980066445	11.96013289	16.61129568	21.59468439	27.90697674	35.54817276	45.18272425	56.47840532	70.09966777	82.72425249	103.3222591	119.6013289	137.8737542	155.8139535	178.7375415	209.3023256	235.8803987	257.807309	275.4152824	293.3554817	300];
  | y_Inconel_718 = [0.576923077	0.892857143	1.826923077	2.513736264	3.186813187	3.846153846	4.450549451	5.068681319	5.645604396	6.195054945	6.634615385	7.225274725	7.596153846	7.93956044	8.228021978	8.516483516	8.818681319	9.07967033	9.299450549	9.491758242	9.725274725	9.848901099];
  | Cond_Inconel_718 =(akima(x_Inconel_718,y_Inconel_718,xt))';
  | x_Hastelloy_X = [4 6.264716558	6.644418163	7.122895706	7.474157486	7.96974	8.407624459	8.917265994	9.457611695	10.1931282	11.04477788	12.09640607	13.10699009	14.50949219	15.89111865	17.4043067	19.16396477	21.32853298	23.6112449	26.27848232	28.62778213	31.69191561	35.27292132	38.42658056	42.31309642	46.84357442	52.69854316	58.6539576	65.28325575	73.83893523	84.41542344	94.96838333	107.9913683	122.8001913	137.4127464	153.7651381	172.0623536	191.5095093	214.2952513	241.0831752	264.0536959	284.6023373	301.8659978];
  | y_Hastelloy_X = [0.7 0.846137913	0.900733102	0.973957115	1.03141131	1.097960859	1.168804371	1.237752699	1.331418781	1.439654868	1.564822259	1.709757645	1.86811709	2.051807187	2.230196716	2.4240959	2.634853191	2.893935687	3.129194704	3.401255144	3.62071366	3.894708671	4.146006192	4.390581075	4.649583548	4.872819029	5.160268949	5.436275753	5.667673067	5.908919904	6.160435512	6.422656985	6.696040023	6.981059723	7.316233877	7.627652383	7.993870698	8.334133095	8.825767583	9.249509722	9.64321891	10.05368649	10.31905456];
  | Cond_Hastelloy_X = (akima(x_Hastelloy_X,y_Hastelloy_X,xt))';
  | 
  | %Cond_4_7 = Cond_Hastelloy_X;
  | Cond_4_7 = Cond_Titanium;
  | 
  | x_heater=[4,65,296];
  | y_heater=[48,49,0];
  | WATTAGE_HEATER=(akima(x_heater,y_heater,xt))';
  | 
  | %Cryocooler algebraic loop parameters
  | TEMP_COLD_HEAD=linspace(2.91,299,2000);
  | x_COLD_HEAD=[2.907692308	4.371428571	5.854945055	6.389010989	7.476923077	15.52747253 18.49148418	20.1946472	21.89781022	23.84428224	25.79075426	27.73722628	29.9270073	32.36009732	34.54987835	37.46958637	40.1459854	43.55231144	46.71532847	49.8783455	52.55474453	55.71776156	58.63746959	61.55717762	64.72019465	67.63990268	70.80291971	74.20924574	77.85888078	81.99513382	85.88807786	89.5377129	93.43065693	97.08029197	100.973236	104.86618	109.7323601	114.5985401	119.2214112	124.8175182	130.4136253	136.4963504	142.8223844	149.3917275	156.9343066	164.7201946	172.5060827	181.0218978	188.8077859	197.56691	206.5693431	214.3552311	221.6545012	230.1703163	238.6861314	248.1751825	257.4209246	265.6934307	273.4793187	281.9951338	292.2141119	299.756691];
  | y_COLD_HEAD=[0	1	1.25	1.5	2	5 5.483870968	6.182795699	6.989247312	7.688172043	8.440860215	9.139784946	9.838709677	10.43010753	11.02150538	11.66666667	12.25806452	12.95698925	13.5483871	14.24731183	14.78494624	15.43010753	16.02150538	16.61290323	17.20430108	17.79569892	18.38709677	18.97849462	19.62365591	20.37634409	21.02150538	21.82795699	22.74193548	23.60215054	24.40860215	25.21505376	26.07526882	26.88172043	27.58064516	28.33333333	28.97849462	29.51612903	29.94623656	30.37634409	30.80645161	31.1827957	31.50537634	31.82795699	32.09677419	32.3655914	32.58064516	32.79569892	33.01075269	33.17204301	33.44086022	33.70967742	33.92473118	34.13978495	34.30107527	34.51612903	34.83870968	35.05376344];
  | WATTAGE_COLD_HEAD=(akima(x_COLD_HEAD,y_COLD_HEAD,TEMP_COLD_HEAD))';
libraries: fl_lib x606, nesl_utility x187, slpidlib x8, simulink x2
(part 1 of 17)
settings Model: Creator=fco17919  LastModifiedBy=lyu87474
settings SolverCC: InitialStep=0.5  MaxConsecutiveMinStep=5  ZeroCrossAlgorithm=Adaptive
settings DebuggingCC: AlgebraicLoopMsg=none  ArtificialAlgebraicLoopMsg=none
settings RTWCC: GPUComputeCapability=3.5
settings SimscapeCC: SimscapeLogType=local  SimscapeLogSimulationStatistics=on  SimscapeLogToSDI=on

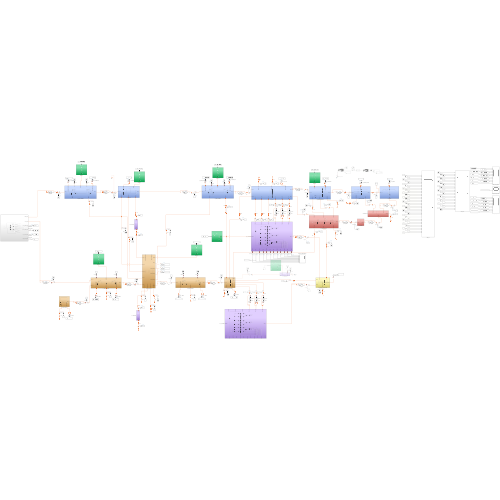
[thumbnail: Simulink's stored preview of the top-level diagram]
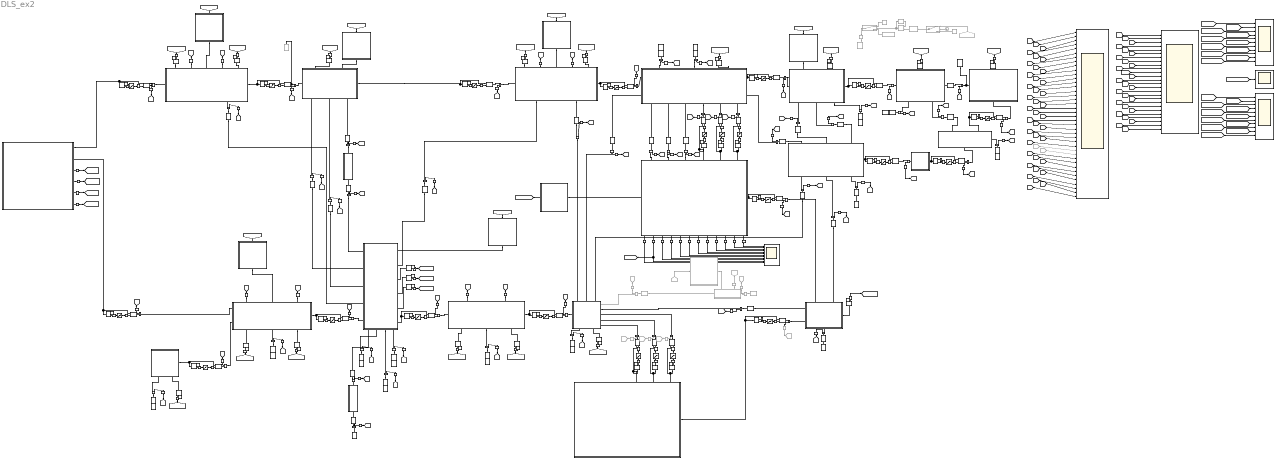
== system DLS_ex2 ==
  1.2_BRAID_ASSEMBLY : Subsystem
      settings: PortSchema="{\"entries\":[{\"content\":{\"sides\":[{\"content\":{\"connectorIds\":[\"LConn1\"]},\"type\":\"ConnectorPlacement.EquallySpacedRectSide\",\"uuid\":\"551ef486-8f55-4086-91e8-3aa1f097044a\"},{\"content\":{\"connectorIds\":[\"RConn1\"],\"side\":\"RIGHT\"},\"type\":\"ConnectorPlacement.EquallySpacedRectSide\",\"uuid\":\"37ccf0f0-295e-42be-80ab-cf5c1c897b82\"},{\"content\":{\"connectorIds\":[\"LConn2\",\"LConn3\",\"LConn4\",\"LConn5\",\"LConn6\"],\"side\":\"TOP\"},\"type\":\"ConnectorPlacement.EquallySpacedRectSide\",\"uuid\":\"69759680-c627-4806-9ba0-7bb938f52c53\"},{\"content\":{\"connectorIds\":[\"RConn2\",\"RConn3\"],\"side\":\"BOTTOM\"},\"type\":\"ConnectorPlacement.EquallySpacedRectSide\",\"uuid\":\"6af0e2fb-4ec0-4d29-999d-afc9a9a00715\"}]},\"type\":\"ConnectorPlacement.EquallySpacedConnector\",\"uuid\":\"48226c00-7a3e-4517-b2a3-8b0a2733c60a\"}],\"packageUris\":[\"http://schema.mathworks.com/mf0/Connector/R2020b\"],\"version\":\"1.0\"}"
  1.3_BUS_BAR : Subsystem
      settings: PortSchema="{\"entries\":[{\"content\":{\"sides\":[{\"content\":{\"connectorIds\":[\"LConn1\"]},\"type\":\"ConnectorPlacement.EquallySpacedRectSide\",\"uuid\":\"25e1045f-0d8f-45fd-a300-cff680178abe\"},{\"content\":{\"connectorIds\":[\"RConn1\"],\"side\":\"RIGHT\"},\"type\":\"ConnectorPlacement.EquallySpacedRectSide\",\"uuid\":\"d29eb369-6963-49ab-ae55-140e7f5d9798\"},{\"content\":{\"connectorIds\":[\"LConn2\",\"LConn3\"],\"side\":\"TOP\"},\"type\":\"ConnectorPlacement.EquallySpacedRectSide\",\"uuid\":\"2759e279-445d-4598-a6af-58d59dd5780f\"},{\"content\":{\"connectorIds\":[\"RConn2\",\"RConn3\",\"RConn4\"],\"side\":\"BOTTOM\"},\"type\":\"ConnectorPlacement.EquallySpacedRectSide\",\"uuid\":\"0c2450c0-eaab-4337-96ae-c46a9e3e2c17\"}]},\"type\":\"ConnectorPlacement.EquallySpacedConnector\",\"uuid\":\"53f3c193-79f5-4556-a40f-c906716c6b3a\"}],\"packageUris\":[\"http://schema.mathworks.com/mf0/Connector/R2020b\"],\"version\":\"1.0\"}"
  1.4_BRAID_ASSEMBLY : Subsystem
      settings: PortSchema="{\"entries\":[{\"content\":{\"sides\":[{\"content\":{\"connectorIds\":[\"LConn1\"]},\"type\":\"ConnectorPlacement.EquallySpacedRectSide\",\"uuid\":\"551ef486-8f55-4086-91e8-3aa1f097044a\"},{\"content\":{\"connectorIds\":[\"RConn1\"],\"side\":\"RIGHT\"},\"type\":\"ConnectorPlacement.EquallySpacedRectSide\",\"uuid\":\"37ccf0f0-295e-42be-80ab-cf5c1c897b82\"},{\"content\":{\"connectorIds\":[\"LConn2\",\"LConn3\",\"LConn4\",\"LConn5\",\"LConn6\"],\"side\":\"TOP\"},\"type\":\"ConnectorPlacement.EquallySpacedRectSide\",\"uuid\":\"69759680-c627-4806-9ba0-7bb938f52c53\"},{\"content\":{\"connectorIds\":[\"RConn2\",\"RConn3\"],\"side\":\"BOTTOM\"},\"type\":\"ConnectorPlacement.EquallySpacedRectSide\",\"uuid\":\"6af0e2fb-4ec0-4d29-999d-afc9a9a00715\"}]},\"type\":\"ConnectorPlacement.EquallySpacedConnector\",\"uuid\":\"48226c00-7a3e-4517-b2a3-8b0a2733c60a\"}],\"packageUris\":[\"http://schema.mathworks.com/mf0/Connector/R2020b\"],\"version\":\"1.0\"}"
  1.5_PULLEY : Subsystem
      settings: PortSchema="{\"entries\":[{\"content\":{\"sides\":[{\"content\":{\"connectorIds\":[\"LConn1\",\"LConn2\"]},\"type\":\"ConnectorPlacement.EquallySpacedRectSide\",\"uuid\":\"25e1045f-0d8f-45fd-a300-cff680178abe\"},{\"content\":{\"connectorIds\":[\"RConn1\",\"RConn2\"],\"side\":\"RIGHT\"},\"type\":\"ConnectorPlacement.EquallySpacedRectSide\",\"uuid\":\"d29eb369-6963-49ab-ae55-140e7f5d9798\"},{\"content\":{\"connectorIds\":[\"LConn3\",\"LConn4\",\"LConn5\"],\"side\":\"TOP\"},\"type\":\"ConnectorPlacement.EquallySpacedRectSide\",\"uuid\":\"2759e279-445d-4598-a6af-58d59dd5780f\"},{\"content\":{\"connectorIds\":[\"RConn3\",\"RConn4\",\"RConn5\",\"RConn6\",\"RConn7\",\"RConn8\"],\"side\":\"BOTTOM\"},\"type\":\"ConnectorPlacement.EquallySpacedRectSide\",\"uuid\":\"0c2450c0-eaab-4337-96ae-c46a9e3e2c17\"}]},\"type\":\"ConnectorPlacement.EquallySpacedConnector\",\"uuid\":\"53f3c193-79f5-4556-a40f-c906716c6b3a\"}],\"packageUris\":[\"http://schema.mathworks.com/mf0/Connector/R2020b\"],\"version\":\"1.0\"}"
  1.6_SAMPLE_RECEIVER : Subsystem
      settings: PortSchema="{\"entries\":[{\"content\":{\"sides\":[{\"content\":{\"connectorIds\":[\"LConn1\"]},\"type\":\"ConnectorPlacement.EquallySpacedRectSide\",\"uuid\":\"25e1045f-0d8f-45fd-a300-cff680178abe\"},{\"content\":{\"connectorIds\":[\"RConn1\"],\"side\":\"RIGHT\"},\"type\":\"ConnectorPlacement.EquallySpacedRectSide\",\"uuid\":\"d29eb369-6963-49ab-ae55-140e7f5d9798\"},{\"content\":{\"connectorIds\":[\"LConn2\",\"LConn3\"],\"side\":\"TOP\"},\"type\":\"ConnectorPlacement.EquallySpacedRectSide\",\"uuid\":\"2759e279-445d-4598-a6af-58d59dd5780f\"},{\"content\":{\"connectorIds\":[\"RConn2\",\"RConn3\",\"RConn4\"],\"side\":\"BOTTOM\"},\"type\":\"ConnectorPlacement.EquallySpacedRectSide\",\"uuid\":\"0c2450c0-eaab-4337-96ae-c46a9e3e2c17\"}]},\"type\":\"ConnectorPlacement.EquallySpacedConnector\",\"uuid\":\"53f3c193-79f5-4556-a40f-c906716c6b3a\"}],\"packageUris\":[\"http://schema.mathworks.com/mf0/Connector/R2020b\"],\"version\":\"1.0\"}"
  1.7_SAMPLE_HOLDER : Subsystem
      settings: PortSchema="{\"entries\":[{\"content\":{\"sides\":[{\"content\":{\"connectorIds\":[\"LConn1\"]},\"type\":\"ConnectorPlacement.EquallySpacedRectSide\",\"uuid\":\"12779b53-17b2-4914-a1e9-059b4fbce4a5\"},{\"content\":{\"connectorIds\":[\"RConn1\"],\"side\":\"RIGHT\"},\"type\":\"ConnectorPlacement.EquallySpacedRectSide\",\"uuid\":\"051696b3-7013-43f2-becf-6a76f1491656\"},{\"content\":{\"connectorIds\":[\"LConn2\"],\"side\":\"TOP\"},\"type\":\"ConnectorPlacement.EquallySpacedRectSide\",\"uuid\":\"1476d0c0-e53e-412a-a5b0-36e6517a2aa9\"},{\"content\":{\"connectorIds\":[\"RConn2\",\"RConn3\"],\"side\":\"BOTTOM\"},\"type\":\"ConnectorPlacement.EquallySpacedRectSide\",\"uuid\":\"cc6ec0bd-f7dd-48cd-bdcb-af2369820998\"}]},\"type\":\"ConnectorPlacement.EquallySpacedConnector\",\"uuid\":\"3b8d0ee5-e4b6-43c8-aa31-01e3bfbfc8de\"}],\"packageUris\":[\"http://schema.mathworks.com/mf0/Connector/R2020b\"],\"version\":\"1.0\"}"
  1.8_SAMPLE : Subsystem
      settings: PortSchema="{\"entries\":[{\"content\":{\"sides\":[{\"content\":{\"connectorIds\":[\"LConn1\"]},\"type\":\"ConnectorPlacement.EquallySpacedRectSide\",\"uuid\":\"73c94150-e284-4f0a-a169-25b222e4ab56\"},{\"content\":{\"side\":\"RIGHT\"},\"type\":\"ConnectorPlacement.EquallySpacedRectSide\",\"uuid\":\"5f321f19-3e25-4427-a9fe-51c433519913\"},{\"content\":{\"connectorIds\":[\"LConn2\"],\"side\":\"TOP\"},\"type\":\"ConnectorPlacement.EquallySpacedRectSide\",\"uuid\":\"c98f79fc-9088-45cf-92c0-0147f3379c8d\"},{\"content\":{\"connectorIds\":[\"RConn1\"],\"side\":\"BOTTOM\"},\"type\":\"ConnectorPlacement.EquallySpacedRectSide\",\"uuid\":\"cec90ba8-5f1b-4109-9dc2-4df0e369925e\"}]},\"type\":\"ConnectorPlacement.EquallySpacedConnector\",\"uuid\":\"5cad9978-3fda-488e-87a0-6e6d92053d40\"}],\"packageUris\":[\"http://schema.mathworks.com/mf0/Connector/R2020b\"],\"version\":\"1.0\"}"
  2.2_RIGID_SHIELD : Subsystem
      settings: PortSchema="{\"entries\":[{\"content\":{\"sides\":[{\"content\":{},\"type\":\"ConnectorPlacement.EquallySpacedRectSide\",\"uuid\":\"e408710b-cacd-4b64-bfc5-fe8d85ab98ae\"},{\"content\":{\"connectorIds\":[\"RConn1\"],\"side\":\"RIGHT\"},\"type\":\"ConnectorPlacement.EquallySpacedRectSide\",\"uuid\":\"a610164c-de9b-4a74-b95f-017fce7b1100\"},{\"content\":{\"side\":\"TOP\"},\"type\":\"ConnectorPlacement.EquallySpacedRectSide\",\"uuid\":\"8a948f38-0b03-47a1-94d5-5a99975ceb5a\"},{\"content\":{\"connectorIds\":[\"RConn2\",\"RConn3\"],\"side\":\"BOTTOM\"},\"type\":\"ConnectorPlacement.EquallySpacedRectSide\",\"uuid\":\"88a61244-f269-43c0-ba9b-49cf4e129ec2\"}]},\"type\":\"ConnectorPlacement.EquallySpacedConnector\",\"uuid\":\"b24256f0-b9c5-440d-8fde-53af2e6c1dbb\"}],\"packageUris\":[\"http://schema.mathworks.com/mf0/Connector/R2020b\"],\"version\":\"1.0\"}"
  2.3_BRAID_ASSEMBLY : Subsystem
      settings: PortSchema="{\"entries\":[{\"content\":{\"sides\":[{\"content\":{\"connectorIds\":[\"LConn1\",\"LConn2\"]},\"type\":\"ConnectorPlacement.EquallySpacedRectSide\",\"uuid\":\"e408710b-cacd-4b64-bfc5-fe8d85ab98ae\"},{\"content\":{\"connectorIds\":[\"RConn1\"],\"side\":\"RIGHT\"},\"type\":\"ConnectorPlacement.EquallySpacedRectSide\",\"uuid\":\"a610164c-de9b-4a74-b95f-017fce7b1100\"},{\"content\":{\"connectorIds\":[\"LConn3\",\"LConn4\",\"LConn5\"],\"side\":\"TOP\"},\"type\":\"ConnectorPlacement.EquallySpacedRectSide\",\"uuid\":\"8a948f38-0b03-47a1-94d5-5a99975ceb5a\"},{\"content\":{\"connectorIds\":[\"RConn2\",\"RConn3\",\"RConn4\"],\"side\":\"BOTTOM\"},\"type\":\"ConnectorPlacement.EquallySpacedRectSide\",\"uuid\":\"88a61244-f269-43c0-ba9b-49cf4e129ec2\"}]},\"type\":\"ConnectorPlacement.EquallySpacedConnector\",\"uuid\":\"b24256f0-b9c5-440d-8fde-53af2e6c1dbb\"}],\"packageUris\":[\"http://schema.mathworks.com/mf0/Connector/R2020b\"],\"version\":\"1.0\"}"
  2.4_RIGID_SHIELD : Subsystem
      settings: PortSchema="{\"entries\":[{\"content\":{\"sides\":[{\"content\":{\"connectorIds\":[\"LConn1\",\"LConn2\",\"LConn3\",\"LConn4\",\"LConn5\"]},\"type\":\"ConnectorPlacement.EquallySpacedRectSide\",\"uuid\":\"e408710b-cacd-4b64-bfc5-fe8d85ab98ae\"},{\"content\":{\"connectorIds\":[\"RConn1\",\"RConn2\",\"RConn3\",\"RConn4\",\"RConn5\",\"RConn6\"],\"side\":\"RIGHT\"},\"type\":\"ConnectorPlacement.EquallySpacedRectSide\",\"uuid\":\"a610164c-de9b-4a74-b95f-017fce7b1100\"},{\"content\":{\"connectorIds\":[\"LConn6\",\"LConn7\"],\"side\":\"TOP\"},\"type\":\"ConnectorPlacement.EquallySpacedRectSide\",\"uuid\":\"8a948f38-0b03-47a1-94d5-5a99975ceb5a\"},{\"content\":{\"connectorIds\":[\"RConn7\",\"RConn8\",\"RConn9\",\"RConn10\"],\"side\":\"BOTTOM\"},\"type\":\"ConnectorPlacement.EquallySpacedRectSide\",\"uuid\":\"88a61244-f269-43c0-ba9b-49cf4e129ec2\"}]},\"type\":\"ConnectorPlacement.EquallySpacedConnector\",\"uuid\":\"b24256f0-b9c5-440d-8fde-53af2e6c1dbb\"}],\"packageUris\":[\"http://schema.mathworks.com/mf0/Connector/R2020b\"],\"version\":\"1.0\"}"
  2.5_BRAID_ASSEMBLY : Subsystem
      settings: PortSchema="{\"entries\":[{\"content\":{\"sides\":[{\"content\":{\"connectorIds\":[\"LConn1\"]},\"type\":\"ConnectorPlacement.EquallySpacedRectSide\",\"uuid\":\"e408710b-cacd-4b64-bfc5-fe8d85ab98ae\"},{\"content\":{\"connectorIds\":[\"RConn1\"],\"side\":\"RIGHT\"},\"type\":\"ConnectorPlacement.EquallySpacedRectSide\",\"uuid\":\"a610164c-de9b-4a74-b95f-017fce7b1100\"},{\"content\":{\"connectorIds\":[\"LConn2\",\"LConn3\"],\"side\":\"TOP\"},\"type\":\"ConnectorPlacement.EquallySpacedRectSide\",\"uuid\":\"8a948f38-0b03-47a1-94d5-5a99975ceb5a\"},{\"content\":{\"connectorIds\":[\"RConn2\",\"RConn3\",\"RConn4\"],\"side\":\"BOTTOM\"},\"type\":\"ConnectorPlacement.EquallySpacedRectSide\",\"uuid\":\"88a61244-f269-43c0-ba9b-49cf4e129ec2\"}]},\"type\":\"ConnectorPlacement.EquallySpacedConnector\",\"uuid\":\"b24256f0-b9c5-440d-8fde-53af2e6c1dbb\"}],\"packageUris\":[\"http://schema.mathworks.com/mf0/Connector/R2020b\"],\"version\":\"1.0\"}"
  2.6_RIGID_SHIELD : Subsystem
      settings: PortSchema="{\"entries\":[{\"content\":{\"sides\":[{\"content\":{\"connectorIds\":[\"LConn1\"]},\"type\":\"ConnectorPlacement.EquallySpacedRectSide\",\"uuid\":\"e408710b-cacd-4b64-bfc5-fe8d85ab98ae\"},{\"content\":{\"connectorIds\":[\"RConn1\",\"RConn2\",\"RConn3\",\"RConn4\",\"RConn5\"],\"side\":\"RIGHT\"},\"type\":\"ConnectorPlacement.EquallySpacedRectSide\",\"uuid\":\"a610164c-de9b-4a74-b95f-017fce7b1100\"},{\"content\":{\"connectorIds\":[\"LConn2\",\"LConn3\",\"LConn4\"],\"side\":\"TOP\"},\"type\":\"ConnectorPlacement.EquallySpacedRectSide\",\"uuid\":\"8a948f38-0b03-47a1-94d5-5a99975ceb5a\"},{\"content\":{\"connectorIds\":[\"RConn6\",\"RConn7\"],\"side\":\"BOTTOM\"},\"type\":\"ConnectorPlacement.EquallySpacedRectSide\",\"uuid\":\"88a61244-f269-43c0-ba9b-49cf4e129ec2\"}]},\"type\":\"ConnectorPlacement.EquallySpacedConnector\",\"uuid\":\"b24256f0-b9c5-440d-8fde-53af2e6c1dbb\"}],\"packageUris\":[\"http://schema.mathworks.com/mf0/Connector/R2020b\"],\"version\":\"1.0\"}"
  3.1_SMARACT_STAGE_ROTARY : Subsystem
      settings: PortSchema="{\"entries\":[{\"content\":{\"sides\":[{\"content\":{\"connectorIds\":[\"LConn1\",\"LConn2\"]},\"type\":\"ConnectorPlacement.EquallySpacedRectSide\",\"uuid\":\"ce9a7825-9424-43e6-aa9d-5c3ea5413f60\"},{\"content\":{\"connectorIds\":[\"RConn1\"],\"side\":\"RIGHT\"},\"type\":\"ConnectorPlacement.EquallySpacedRectSide\",\"uuid\":\"40fd49ee-49a7-447c-9616-f7c6d2963d6d\"},{\"content\":{\"connectorIds\":[\"LConn3\",\"LConn4\"],\"side\":\"TOP\"},\"type\":\"ConnectorPlacement.EquallySpacedRectSide\",\"uuid\":\"ab940ee3-335f-46f7-ab56-b94d696c7ed8\"},{\"content\":{\"connectorIds\":[\"RConn2\"],\"side\":\"BOTTOM\"},\"type\":\"ConnectorPlacement.EquallySpacedRectSide\",\"uuid\":\"174f2bab-6efc-40a7-a499-c7960d69d571\"}]},\"type\":\"ConnectorPlacement.EquallySpacedConnector\",\"uuid\":\"7f8076d6-e925-4f60-8d1a-e96761ed5822\"}],\"packageUris\":[\"http://schema.mathworks.com/mf0/Connector/R2020b\"],\"version\":\"1.0\"}"
  4.2_INSULATOR : Subsystem
  4.3_INSULATOR : Subsystem
  4.4_INSULATOR : Subsystem  Commented=on
      settings: PortSchema="{\"entries\":[{\"content\":{\"sides\":[{\"content\":{\"connectorIds\":[\"LConn1\"]},\"type\":\"ConnectorPlacement.EquallySpacedRectSide\",\"uuid\":\"a4b6422d-954e-4ffa-b410-aa2b5aade717\"},{\"content\":{\"connectorIds\":[\"RConn1\"],\"side\":\"RIGHT\"},\"type\":\"ConnectorPlacement.EquallySpacedRectSide\",\"uuid\":\"7da939f4-5bc8-4776-872b-27edefe2e831\"},{\"content\":{\"connectorIds\":[\"LConn2\",\"LConn3\"],\"side\":\"TOP\"},\"type\":\"ConnectorPlacement.EquallySpacedRectSide\",\"uuid\":\"e2bf41db-ef5d-46a6-857e-e03fa9448ec6\"}]},\"type\":\"ConnectorPlacement.EquallySpacedConnector\",\"uuid\":\"dfeda41b-5461-4c65-b1ec-0b80e8653652\"}],\"packageUris\":[\"http://schema.mathworks.com/mf0/Connector/R2020b\"],\"version\":\"1.0\"}"
  4.7_TI_FLEXURE : Subsystem
      settings: PortSchema="{\"entries\":[{\"content\":{\"sides\":[{\"content\":{\"connectorIds\":[\"LConn1\"]},\"type\":\"ConnectorPlacement.EquallySpacedRectSide\",\"uuid\":\"d5efd99e-a0bc-4485-99e2-6f4ace98708f\"},{\"content\":{\"connectorIds\":[\"RConn1\"],\"side\":\"RIGHT\"},\"type\":\"ConnectorPlacement.EquallySpacedRectSide\",\"uuid\":\"9db6695c-6692-4d0b-9b11-5f5ada9fd794\"},{\"content\":{\"connectorIds\":[\"LConn2\",\"LConn3\",\"LConn4\",\"LConn5\",\"LConn6\",\"LConn7\"],\"side\":\"TOP\"},\"type\":\"ConnectorPlacement.EquallySpacedRectSide\",\"uuid\":\"4c2aa0bd-aa80-4661-b1d3-39b0266186fa\"},{\"content\":{\"connectorIds\":[\"RConn2\",\"RConn3\",\"RConn4\",\"RConn5\",\"RConn6\",\"RConn7\",\"RConn8\",\"RConn9\",\"RConn10\",\"RConn11\",\"RConn12\",\"RConn13\"],\"side\":\"BOTTOM\"},\"type\":\"ConnectorPlacement.EquallySpacedRectSide\",\"uuid\":\"59fe0495-b79b-4f0d-b2e5-736358fa0893\"}]},\"type\":\"ConnectorPlacement.EquallySpacedConnector\",\"uuid\":\"4b6fc19e-32b8-48c0-81a2-016cf691ff70\"}],\"packageUris\":[\"http://schema.mathworks.com/mf0/Connector/R2020b\"],\"version\":\"1.0\"}"
  4.7_TI_FLEXURE1 : Subsystem
      settings: PortSchema="{\"entries\":[{\"content\":{\"sides\":[{\"content\":{\"connectorIds\":[\"LConn1\"]},\"type\":\"ConnectorPlacement.EquallySpacedRectSide\",\"uuid\":\"d5efd99e-a0bc-4485-99e2-6f4ace98708f\"},{\"content\":{\"connectorIds\":[\"RConn1\"],\"side\":\"RIGHT\"},\"type\":\"ConnectorPlacement.EquallySpacedRectSide\",\"uuid\":\"9db6695c-6692-4d0b-9b11-5f5ada9fd794\"},{\"content\":{\"connectorIds\":[\"LConn2\",\"LConn3\",\"LConn4\",\"LConn5\",\"LConn6\",\"LConn7\"],\"side\":\"TOP\"},\"type\":\"ConnectorPlacement.EquallySpacedRectSide\",\"uuid\":\"4c2aa0bd-aa80-4661-b1d3-39b0266186fa\"},{\"content\":{\"connectorIds\":[\"RConn2\",\"RConn3\",\"RConn4\",\"RConn5\",\"RConn6\",\"RConn7\",\"RConn8\",\"RConn9\",\"RConn10\",\"RConn11\",\"RConn12\",\"RConn13\"],\"side\":\"BOTTOM\"},\"type\":\"ConnectorPlacement.EquallySpacedRectSide\",\"uuid\":\"59fe0495-b79b-4f0d-b2e5-736358fa0893\"}]},\"type\":\"ConnectorPlacement.EquallySpacedConnector\",\"uuid\":\"4b6fc19e-32b8-48c0-81a2-016cf691ff70\"}],\"packageUris\":[\"http://schema.mathworks.com/mf0/Connector/R2020b\"],\"version\":\"1.0\"}"
  7.1 CABLE ASSEMBLY : Subsystem
      settings: PortSchema="{\"entries\":[{\"content\":{\"sides\":[{\"content\":{},\"type\":\"ConnectorPlacement.EquallySpacedRectSide\",\"uuid\":\"e408710b-cacd-4b64-bfc5-fe8d85ab98ae\"},{\"content\":{\"connectorIds\":[\"RConn1\"],\"side\":\"RIGHT\"},\"type\":\"ConnectorPlacement.EquallySpacedRectSide\",\"uuid\":\"a610164c-de9b-4a74-b95f-017fce7b1100\"},{\"content\":{\"connectorIds\":[\"LConn1\",\"LConn2\",\"LConn3\"],\"side\":\"TOP\"},\"type\":\"ConnectorPlacement.EquallySpacedRectSide\",\"uuid\":\"8a948f38-0b03-47a1-94d5-5a99975ceb5a\"},{\"content\":{\"connectorIds\":[\"RConn2\",\"RConn3\",\"RConn4\"],\"side\":\"BOTTOM\"},\"type\":\"ConnectorPlacement.EquallySpacedRectSide\",\"uuid\":\"88a61244-f269-43c0-ba9b-49cf4e129ec2\"}]},\"type\":\"ConnectorPlacement.EquallySpacedConnector\",\"uuid\":\"b24256f0-b9c5-440d-8fde-53af2e6c1dbb\"}],\"packageUris\":[\"http://schema.mathworks.com/mf0/Connector/R2020b\"],\"version\":\"1.0\"}"
  7.3 PCB PINS : Subsystem
  7.4 SAMPLE PCB : Subsystem
      settings: PortSchema="{\"entries\":[{\"content\":{\"sides\":[{\"content\":{},\"type\":\"ConnectorPlacement.EquallySpacedRectSide\",\"uuid\":\"3626635b-af14-4108-b396-c389795bd8b7\"},{\"content\":{\"connectorIds\":[\"RConn1\"],\"side\":\"RIGHT\"},\"type\":\"ConnectorPlacement.EquallySpacedRectSide\",\"uuid\":\"9c71ba38-7144-4bd6-a713-cd6b78f8286b\"},{\"content\":{\"connectorIds\":[\"LConn1\",\"LConn2\"],\"side\":\"TOP\"},\"type\":\"ConnectorPlacement.EquallySpacedRectSide\",\"uuid\":\"57e9682b-af26-429d-84aa-a88d4aea0a7f\"},{\"content\":{\"connectorIds\":[\"RConn2\"],\"side\":\"BOTTOM\"},\"type\":\"ConnectorPlacement.EquallySpacedRectSide\",\"uuid\":\"3a789ba0-835f-4dbb-8a9b-8120076ae74a\"}]},\"type\":\"ConnectorPlacement.EquallySpacedConnector\",\"uuid\":\"6ccaac5f-b17f-4a55-a02f-ce876d53679b\"}],\"packageUris\":[\"http://schema.mathworks.com/mf0/Connector/R2020b\"],\"version\":\"1.0\"}"
  A{1..2,4..5,8..10,12,14..15,20..21,24..25,28,38} (16 alike) : fl_lib/Thermal/Thermal Elements/Variable Thermal Resistance  R_min=0 K/W  T_specify=off  T_priority=None  T=0 K  T_nominal_specify=off  T_nominal_value=1  T_nominal_unit=K  Q_specify=off  Q_priority=None  Q=0 W  Q_nominal_specify=off  Q_nominal_value=1  Q_nominal_unit=W
      settings: InternalSimscapePortConfiguration="{\"Bottom\":[],\"Left\":[{\"id\":\"A\",\"label\":\"A\",\"type\":\"foundation.thermal.thermal\"},{\"id\":\"R\",\"label\":\"R\",\"type\":\"input\"}],\"Right\":[{\"id\":\"B\",\"label\":\"B\",\"type\":\"foundation.thermal.thermal\"}],\"Top\":[]}"
  A11 : fl_lib/Thermal/Thermal Elements/Thermal Resistance  resistance=res_A11 K/W  T_specify=off  T_priority=None  T=0 K  T_nominal_specify=off  T_nominal_value=1  T_nominal_unit=K  Q_specify=off  Q_priority=None  Q=0 W  Q_nominal_specify=off  Q_nominal_value=1  Q_nominal_unit=W
  A13 : fl_lib/Thermal/Thermal Elements/Thermal Resistance  resistance=res_A17 K/W  T_specify=off  T_priority=None  T=0 K  T_nominal_specify=off  T_nominal_value=1  T_nominal_unit=K  Q_specify=off  Q_priority=None  Q=0 W  Q_nominal_specify=off  Q_nominal_value=1  Q_nominal_unit=W
  A16 : fl_lib/Thermal/Thermal Elements/Thermal Resistance  resistance=res_A17 K/W  T_specify=off  T_priority=None  T=0 K  T_nominal_specify=off  T_nominal_value=1  T_nominal_unit=K  Q_specify=off  Q_priority=None  Q=0 W  Q_nominal_specify=off  Q_nominal_value=1  Q_nominal_unit=W
  A17 : fl_lib/Thermal/Thermal Elements/Thermal Resistance  Commented=on  resistance=res_A17 K/W  T_specify=off  T_priority=None  T=0 K  T_nominal_specify=off  T_nominal_value=1  T_nominal_unit=K  Q_specify=off  Q_priority=None  Q=0 W  Q_nominal_specify=off  Q_nominal_value=1  Q_nominal_unit=W
  A18 : fl_lib/Thermal/Thermal Elements/Thermal Resistance  Commented=on  resistance=res_A18 K/W  T_specify=off  T_priority=None  T=0 K  T_nominal_specify=off  T_nominal_value=1  T_nominal_unit=K  Q_specify=off  Q_priority=None  Q=0 W  Q_nominal_specify=off  Q_nominal_value=1  Q_nominal_unit=W
  A19 : fl_lib/Thermal/Thermal Elements/Thermal Resistance  resistance=res_A19 K/W  T_specify=off  T_priority=None  T=0 K  T_nominal_specify=off  T_nominal_value=1  T_nominal_unit=K  Q_specify=off  Q_priority=None  Q=0 W  Q_nominal_specify=off  Q_nominal_value=1  Q_nominal_unit=W
  A31 : fl_lib/Thermal/Thermal Elements/Thermal Resistance  resistance=res_A31 K/W  T_specify=off  T_priority=None  T=0 K  T_nominal_specify=off  T_nominal_value=1  T_nominal_unit=K  Q_specify=off  Q_priority=None  Q=0 W  Q_nominal_specify=off  Q_nominal_value=1  Q_nominal_unit=W
  A32 : fl_lib/Thermal/Thermal Elements/Thermal Resistance  resistance=res_A32 K/W  T_specify=off  T_priority=None  T=0 K  T_nominal_specify=off  T_nominal_value=1  T_nominal_unit=K  Q_specify=off  Q_priority=None  Q=0 W  Q_nominal_specify=off  Q_nominal_value=1  Q_nominal_unit=W
  A33 : fl_lib/Thermal/Thermal Elements/Thermal Resistance  resistance=res_A33 K/W  T_specify=off  T_priority=None  T=0 K  T_nominal_specify=off  T_nominal_value=1  T_nominal_unit=K  Q_specify=off  Q_priority=None  Q=0 W  Q_nominal_specify=off  Q_nominal_value=1  Q_nominal_unit=W
  A34 : fl_lib/Thermal/Thermal Elements/Thermal Resistance  resistance=res_A34 K/W  T_specify=off  T_priority=None  T=0 K  T_nominal_specify=off  T_nominal_value=1  T_nominal_unit=K  Q_specify=off  Q_priority=None  Q=0 W  Q_nominal_specify=off  Q_nominal_value=1  Q_nominal_unit=W
  A36 : fl_lib/Thermal/Thermal Elements/Thermal Resistance  resistance=res_A36 K/W  T_specify=off  T_priority=None  T=0 K  T_nominal_specify=off  T_nominal_value=1  T_nominal_unit=K  Q_specify=off  Q_priority=None  Q=0 W  Q_nominal_specify=off  Q_nominal_value=1  Q_nominal_unit=W
  A37.{1..6} (6 alike) : fl_lib/Thermal/Thermal Elements/Variable Thermal Resistance  R_min=0 K/W  T_specify=off  T_priority=None  T=0 K  T_nominal_specify=off  T_nominal_value=1  T_nominal_unit=K  Q_specify=off  Q_priority=None  Q=0 W  Q_nominal_specify=off  Q_nominal_value=1  Q_nominal_unit=W
      settings: InternalSimscapePortConfiguration="{\"Bottom\":[],\"Left\":[{\"id\":\"A\",\"label\":\"A\",\"type\":\"foundation.thermal.thermal\"},{\"id\":\"R\",\"label\":\"R\",\"type\":\"input\"}],\"Right\":[{\"id\":\"B\",\"label\":\"B\",\"type\":\"foundation.thermal.thermal\"}],\"Top\":[]}"
  B1 : fl_lib/Thermal/Thermal Elements/Radiative Heat Transfer  area=Area_B1 mm^2  rad_tr_coeff=K_B1 W/(K^4*m^2)  T_specify=off  T_priority=None  T=0 K  T_nominal_specify=off  T_nominal_value=1  T_nominal_unit=K  Q_specify=off  Q_priority=None  Q=0 W  Q_nominal_specify=off  Q_nominal_value=1  Q_nominal_unit=W
      settings: InternalSimscapePortConfiguration="{\"Bottom\":[],\"Left\":[{\"id\":\"A\",\"label\":\"A\",\"type\":\"foundation.thermal.thermal\"}],\"Right\":[{\"id\":\"B\",\"label\":\"B\",\"type\":\"foundation.thermal.thermal\"}],\"Top\":[]}"
  B10.1 : fl_lib/Thermal/Thermal Elements/Radiative Heat Transfer  area=Area_B10 mm^2  rad_tr_coeff=K_B10 W/(K^4*m^2)  T_specify=off  T_priority=None  T=0 K  T_nominal_specify=off  T_nominal_value=1  T_nominal_unit=K  Q_specify=off  Q_priority=None  Q=0 W  Q_nominal_specify=off  Q_nominal_value=1  Q_nominal_unit=W
      settings: InternalSimscapePortConfiguration="{\"Bottom\":[],\"Left\":[{\"id\":\"A\",\"label\":\"A\",\"type\":\"foundation.thermal.thermal\"}],\"Right\":[{\"id\":\"B\",\"label\":\"B\",\"type\":\"foundation.thermal.thermal\"}],\"Top\":[]}"
  B10.2 : fl_lib/Thermal/Thermal Elements/Radiative Heat Transfer  area=Area_B10 mm^2  rad_tr_coeff=K_B10 W/(K^4*m^2)  T_specify=off  T_priority=None  T=0 K  T_nominal_specify=off  T_nominal_value=1  T_nominal_unit=K  Q_specify=off  Q_priority=None  Q=0 W  Q_nominal_specify=off  Q_nominal_value=1  Q_nominal_unit=W
      settings: InternalSimscapePortConfiguration="{\"Bottom\":[],\"Left\":[{\"id\":\"A\",\"label\":\"A\",\"type\":\"foundation.thermal.thermal\"}],\"Right\":[{\"id\":\"B\",\"label\":\"B\",\"type\":\"foundation.thermal.thermal\"}],\"Top\":[]}"
  B10.3 : fl_lib/Thermal/Thermal Elements/Radiative Heat Transfer  area=Area_B10 mm^2  rad_tr_coeff=K_B10 W/(K^4*m^2)  T_specify=off  T_priority=None  T=0 K  T_nominal_specify=off  T_nominal_value=1  T_nominal_unit=K  Q_specify=off  Q_priority=None  Q=0 W  Q_nominal_specify=off  Q_nominal_value=1  Q_nominal_unit=W
      settings: InternalSimscapePortConfiguration="{\"Bottom\":[],\"Left\":[{\"id\":\"A\",\"label\":\"A\",\"type\":\"foundation.thermal.thermal\"}],\"Right\":[{\"id\":\"B\",\"label\":\"B\",\"type\":\"foundation.thermal.thermal\"}],\"Top\":[]}"
  B13 : fl_lib/Thermal/Thermal Elements/Radiative Heat Transfer  area=Area_B13 mm^2  rad_tr_coeff=K_B13 W/(K^4*m^2)  T_specify=off  T_priority=None  T=0 K  T_nominal_specify=off  T_nominal_value=1  T_nominal_unit=K  Q_specify=off  Q_priority=None  Q=0 W  Q_nominal_specify=off  Q_nominal_value=1  Q_nominal_unit=W
      settings: InternalSimscapePortConfiguration="{\"Bottom\":[],\"Left\":[{\"id\":\"A\",\"label\":\"A\",\"type\":\"foundation.thermal.thermal\"}],\"Right\":[{\"id\":\"B\",\"label\":\"B\",\"type\":\"foundation.thermal.thermal\"}],\"Top\":[]}"
  B14 : fl_lib/Thermal/Thermal Elements/Radiative Heat Transfer  area=Area_B14 mm^2  rad_tr_coeff=K_B14 W/(K^4*m^2)  T_specify=off  T_priority=None  T=0 K  T_nominal_specify=off  T_nominal_value=1  T_nominal_unit=K  Q_specify=off  Q_priority=None  Q=0 W  Q_nominal_specify=off  Q_nominal_value=1  Q_nominal_unit=W
      settings: InternalSimscapePortConfiguration="{\"Bottom\":[],\"Left\":[{\"id\":\"A\",\"label\":\"A\",\"type\":\"foundation.thermal.thermal\"}],\"Right\":[{\"id\":\"B\",\"label\":\"B\",\"type\":\"foundation.thermal.thermal\"}],\"Top\":[]}"
  B15 : fl_lib/Thermal/Thermal Elements/Radiative Heat Transfer  area=Area_B15 mm^2  rad_tr_coeff=K_B15 W/(K^4*m^2)  T_specify=off  T_priority=None  T=0 K  T_nominal_specify=off  T_nominal_value=1  T_nominal_unit=K  Q_specify=off  Q_priority=None  Q=0 W  Q_nominal_specify=off  Q_nominal_value=1  Q_nominal_unit=W
      settings: InternalSimscapePortConfiguration="{\"Bottom\":[],\"Left\":[{\"id\":\"A\",\"label\":\"A\",\"type\":\"foundation.thermal.thermal\"}],\"Right\":[{\"id\":\"B\",\"label\":\"B\",\"type\":\"foundation.thermal.thermal\"}],\"Top\":[]}"
  B16 : fl_lib/Thermal/Thermal Elements/Radiative Heat Transfer  area=Area_B16 mm^2  rad_tr_coeff=K_B16 W/(K^4*m^2)  T_specify=off  T_priority=None  T=0 K  T_nominal_specify=off  T_nominal_value=1  T_nominal_unit=K  Q_specify=off  Q_priority=None  Q=0 W  Q_nominal_specify=off  Q_nominal_value=1  Q_nominal_unit=W
      settings: InternalSimscapePortConfiguration="{\"Bottom\":[],\"Left\":[{\"id\":\"A\",\"label\":\"A\",\"type\":\"foundation.thermal.thermal\"}],\"Right\":[{\"id\":\"B\",\"label\":\"B\",\"type\":\"foundation.thermal.thermal\"}],\"Top\":[]}"
  B17 : fl_lib/Thermal/Thermal Elements/Radiative Heat Transfer  area=Area_B17 mm^2  rad_tr_coeff=K_B17 W/(K^4*m^2)  T_specify=off  T_priority=None  T=0 K  T_nominal_specify=off  T_nominal_value=1  T_nominal_unit=K  Q_specify=off  Q_priority=None  Q=0 W  Q_nominal_specify=off  Q_nominal_value=1  Q_nominal_unit=W
      settings: InternalSimscapePortConfiguration="{\"Bottom\":[],\"Left\":[{\"id\":\"A\",\"label\":\"A\",\"type\":\"foundation.thermal.thermal\"}],\"Right\":[{\"id\":\"B\",\"label\":\"B\",\"type\":\"foundation.thermal.thermal\"}],\"Top\":[]}"
  B18 : fl_lib/Thermal/Thermal Elements/Radiative Heat Transfer  area=Area_B18 mm^2  rad_tr_coeff=K_B18 W/(K^4*m^2)  T_specify=off  T_priority=None  T=0 K  T_nominal_specify=off  T_nominal_value=1  T_nominal_unit=K  Q_specify=off  Q_priority=None  Q=0 W  Q_nominal_specify=off  Q_nominal_value=1  Q_nominal_unit=W
      settings: InternalSimscapePortConfiguration="{\"Bottom\":[],\"Left\":[{\"id\":\"A\",\"label\":\"A\",\"type\":\"foundation.thermal.thermal\"}],\"Right\":[{\"id\":\"B\",\"label\":\"B\",\"type\":\"foundation.thermal.thermal\"}],\"Top\":[]}"
  B19 : fl_lib/Thermal/Thermal Elements/Radiative Heat Transfer  area=Area_B19 mm^2  rad_tr_coeff=K_B19 W/(K^4*m^2)  T_specify=off  T_priority=None  T=0 K  T_nominal_specify=off  T_nominal_value=1  T_nominal_unit=K  Q_specify=off  Q_priority=None  Q=0 W  Q_nominal_specify=off  Q_nominal_value=1  Q_nominal_unit=W
      settings: InternalSimscapePortConfiguration="{\"Bottom\":[],\"Left\":[{\"id\":\"A\",\"label\":\"A\",\"type\":\"foundation.thermal.thermal\"}],\"Right\":[{\"id\":\"B\",\"label\":\"B\",\"type\":\"foundation.thermal.thermal\"}],\"Top\":[]}"
  B2 : fl_lib/Thermal/Thermal Elements/Radiative Heat Transfer  area=Area_B2 mm^2  rad_tr_coeff=K_B2 W/(K^4*m^2)  T_specify=off  T_priority=None  T=0 K  T_nominal_specify=off  T_nominal_value=1  T_nominal_unit=K  Q_specify=off  Q_priority=None  Q=0 W  Q_nominal_specify=off  Q_nominal_value=1  Q_nominal_unit=W
      settings: InternalSimscapePortConfiguration="{\"Bottom\":[],\"Left\":[{\"id\":\"A\",\"label\":\"A\",\"type\":\"foundation.thermal.thermal\"}],\"Right\":[{\"id\":\"B\",\"label\":\"B\",\"type\":\"foundation.thermal.thermal\"}],\"Top\":[]}"
  B20 : fl_lib/Thermal/Thermal Elements/Radiative Heat Transfer  area=Area_B20 mm^2  rad_tr_coeff=K_B20 W/(K^4*m^2)  T_specify=off  T_priority=None  T=0 K  T_nominal_specify=off  T_nominal_value=1  T_nominal_unit=K  Q_specify=off  Q_priority=None  Q=0 W  Q_nominal_specify=off  Q_nominal_value=1  Q_nominal_unit=W
      settings: InternalSimscapePortConfiguration="{\"Bottom\":[],\"Left\":[{\"id\":\"A\",\"label\":\"A\",\"type\":\"foundation.thermal.thermal\"}],\"Right\":[{\"id\":\"B\",\"label\":\"B\",\"type\":\"foundation.thermal.thermal\"}],\"Top\":[]}"
  B21 : fl_lib/Thermal/Thermal Elements/Radiative Heat Transfer  area=Area_B21 mm^2  rad_tr_coeff=K_B21 W/(K^4*m^2)  T_specify=off  T_priority=None  T=0 K  T_nominal_specify=off  T_nominal_value=1  T_nominal_unit=K  Q_specify=off  Q_priority=None  Q=0 W  Q_nominal_specify=off  Q_nominal_value=1  Q_nominal_unit=W
      settings: InternalSimscapePortConfiguration="{\"Bottom\":[],\"Left\":[{\"id\":\"A\",\"label\":\"A\",\"type\":\"foundation.thermal.thermal\"}],\"Right\":[{\"id\":\"B\",\"label\":\"B\",\"type\":\"foundation.thermal.thermal\"}],\"Top\":[]}"
  B22 : fl_lib/Thermal/Thermal Elements/Radiative Heat Transfer  area=Area_B22 mm^2  rad_tr_coeff=K_B22 W/(K^4*m^2)  T_specify=off  T_priority=None  T=0 K  T_nominal_specify=off  T_nominal_value=1  T_nominal_unit=K  Q_specify=off  Q_priority=None  Q=0 W  Q_nominal_specify=off  Q_nominal_value=1  Q_nominal_unit=W
      settings: InternalSimscapePortConfiguration="{\"Bottom\":[],\"Left\":[{\"id\":\"A\",\"label\":\"A\",\"type\":\"foundation.thermal.thermal\"}],\"Right\":[{\"id\":\"B\",\"label\":\"B\",\"type\":\"foundation.thermal.thermal\"}],\"Top\":[]}"
  B23 : fl_lib/Thermal/Thermal Elements/Radiative Heat Transfer  area=Area_B23 mm^2  rad_tr_coeff=K_B23 W/(K^4*m^2)  T_specify=off  T_priority=None  T=0 K  T_nominal_specify=off  T_nominal_value=1  T_nominal_unit=K  Q_specify=off  Q_priority=None  Q=0 W  Q_nominal_specify=off  Q_nominal_value=1  Q_nominal_unit=W
      settings: InternalSimscapePortConfiguration="{\"Bottom\":[],\"Left\":[{\"id\":\"A\",\"label\":\"A\",\"type\":\"foundation.thermal.thermal\"}],\"Right\":[{\"id\":\"B\",\"label\":\"B\",\"type\":\"foundation.thermal.thermal\"}],\"Top\":[]}"
  B25 : fl_lib/Thermal/Thermal Elements/Radiative Heat Transfer  area=Area_B25 mm^2  rad_tr_coeff=K_B25 W/(K^4*m^2)  T_specify=off  T_priority=None  T=0 K  T_nominal_specify=off  T_nominal_value=1  T_nominal_unit=K  Q_specify=off  Q_priority=None  Q=0 W  Q_nominal_specify=off  Q_nominal_value=1  Q_nominal_unit=W
      settings: InternalSimscapePortConfiguration="{\"Bottom\":[],\"Left\":[{\"id\":\"A\",\"label\":\"A\",\"type\":\"foundation.thermal.thermal\"}],\"Right\":[{\"id\":\"B\",\"label\":\"B\",\"type\":\"foundation.thermal.thermal\"}],\"Top\":[]}"
  B26 : fl_lib/Thermal/Thermal Elements/Radiative Heat Transfer  area=2557*2/3 mm^2  rad_tr_coeff=|  T_specify=off  T_priority=None  T=0 K  T_nominal_specify=off  T_nominal_value=1  T_nominal_unit=K  Q_specify=off  Q_priority=None  Q=0 W  Q_nominal_specify=off  Q_nominal_value=1  Q_nominal_unit=W
      | 1.08E-08
      |  W/(K^4*m^2)
      settings: InternalSimscapePortConfiguration="{\"Bottom\":[],\"Left\":[{\"id\":\"A\",\"label\":\"A\",\"type\":\"foundation.thermal.thermal\"}],\"Right\":[{\"id\":\"B\",\"label\":\"B\",\"type\":\"foundation.thermal.thermal\"}],\"Top\":[]}"
  B27 : fl_lib/Thermal/Thermal Elements/Radiative Heat Transfer  area=2557/3 mm^2  rad_tr_coeff=|  T_specify=off  T_priority=None  T=0 K  T_nominal_specify=off  T_nominal_value=1  T_nominal_unit=K  Q_specify=off  Q_priority=None  Q=0 W  Q_nominal_specify=off  Q_nominal_value=1  Q_nominal_unit=W
      | 1.08E-08
      |  W/(K^4*m^2)
      settings: InternalSimscapePortConfiguration="{\"Bottom\":[],\"Left\":[{\"id\":\"A\",\"label\":\"A\",\"type\":\"foundation.thermal.thermal\"}],\"Right\":[{\"id\":\"B\",\"label\":\"B\",\"type\":\"foundation.thermal.thermal\"}],\"Top\":[]}"
  B3 : fl_lib/Thermal/Thermal Elements/Radiative Heat Transfer  area=Area_B3 mm^2  rad_tr_coeff=K_B3 W/(K^4*m^2)  T_specify=off  T_priority=None  T=0 K  T_nominal_specify=off  T_nominal_value=1  T_nominal_unit=K  Q_specify=off  Q_priority=None  Q=0 W  Q_nominal_specify=off  Q_nominal_value=1  Q_nominal_unit=W
      settings: InternalSimscapePortConfiguration="{\"Bottom\":[],\"Left\":[{\"id\":\"A\",\"label\":\"A\",\"type\":\"foundation.thermal.thermal\"}],\"Right\":[{\"id\":\"B\",\"label\":\"B\",\"type\":\"foundation.thermal.thermal\"}],\"Top\":[]}"
  B4 : fl_lib/Thermal/Thermal Elements/Radiative Heat Transfer  area=Area_B4 mm^2  rad_tr_coeff=K_B4 W/(K^4*m^2)  T_specify=off  T_priority=None  T=0 K  T_nominal_specify=off  T_nominal_value=1  T_nominal_unit=K  Q_specify=off  Q_priority=None  Q=0 W  Q_nominal_specify=off  Q_nominal_value=1  Q_nominal_unit=W
      settings: InternalSimscapePortConfiguration="{\"Bottom\":[],\"Left\":[{\"id\":\"A\",\"label\":\"A\",\"type\":\"foundation.thermal.thermal\"}],\"Right\":[{\"id\":\"B\",\"label\":\"B\",\"type\":\"foundation.thermal.thermal\"}],\"Top\":[]}"
  B5 : fl_lib/Thermal/Thermal Elements/Radiative Heat Transfer  area=Area_B5 mm^2  rad_tr_coeff=K_B5/2 W/(K^4*m^2)  T_specify=off  T_priority=None  T=0 K  T_nominal_specify=off  T_nominal_value=1  T_nominal_unit=K  Q_specify=off  Q_priority=None  Q=0 W  Q_nominal_specify=off  Q_nominal_value=1  Q_nominal_unit=W
      settings: InternalSimscapePortConfiguration="{\"Bottom\":[],\"Left\":[{\"id\":\"A\",\"label\":\"A\",\"type\":\"foundation.thermal.thermal\"}],\"Right\":[{\"id\":\"B\",\"label\":\"B\",\"type\":\"foundation.thermal.thermal\"}],\"Top\":[]}"
  B6 : fl_lib/Thermal/Thermal Elements/Radiative Heat Transfer  area=Area_B6 mm^2  rad_tr_coeff=K_B6/2 W/(K^4*m^2)  T_specify=off  T_priority=None  T=0 K  T_nominal_specify=off  T_nominal_value=1  T_nominal_unit=K  Q_specify=off  Q_priority=None  Q=0 W  Q_nominal_specify=off  Q_nominal_value=1  Q_nominal_unit=W
      settings: InternalSimscapePortConfiguration="{\"Bottom\":[],\"Left\":[{\"id\":\"A\",\"label\":\"A\",\"type\":\"foundation.thermal.thermal\"}],\"Right\":[{\"id\":\"B\",\"label\":\"B\",\"type\":\"foundation.thermal.thermal\"}],\"Top\":[]}"
  B7 : fl_lib/Thermal/Thermal Elements/Radiative Heat Transfer  area=Area_B7 mm^2  rad_tr_coeff=K_B7 W/(K^4*m^2)  T_specify=off  T_priority=None  T=0 K  T_nominal_specify=off  T_nominal_value=1  T_nominal_unit=K  Q_specify=off  Q_priority=None  Q=0 W  Q_nominal_specify=off  Q_nominal_value=1  Q_nominal_unit=W
      settings: InternalSimscapePortConfiguration="{\"Bottom\":[],\"Left\":[{\"id\":\"A\",\"label\":\"A\",\"type\":\"foundation.thermal.thermal\"}],\"Right\":[{\"id\":\"B\",\"label\":\"B\",\"type\":\"foundation.thermal.thermal\"}],\"Top\":[]}"
  B8 : fl_lib/Thermal/Thermal Elements/Radiative Heat Transfer  area=Area_B8 mm^2  rad_tr_coeff=K_B8 W/(K^4*m^2)  T_specify=off  T_priority=None  T=0 K  T_nominal_specify=off  T_nominal_value=1  T_nominal_unit=K  Q_specify=off  Q_priority=None  Q=0 W  Q_nominal_specify=off  Q_nominal_value=1  Q_nominal_unit=W
      settings: InternalSimscapePortConfiguration="{\"Bottom\":[],\"Left\":[{\"id\":\"A\",\"label\":\"A\",\"type\":\"foundation.thermal.thermal\"}],\"Right\":[{\"id\":\"B\",\"label\":\"B\",\"type\":\"foundation.thermal.thermal\"}],\"Top\":[]}"
  B9 : fl_lib/Thermal/Thermal Elements/Radiative Heat Transfer  area=Area_B9 mm^2  rad_tr_coeff=K_B9 W/(K^4*m^2)  T_specify=off  T_priority=None  T=0 K  T_nominal_specify=off  T_nominal_value=1  T_nominal_unit=K  Q_specify=off  Q_priority=None  Q=0 W  Q_nominal_specify=off  Q_nominal_value=1  Q_nominal_unit=W
      settings: InternalSimscapePortConfiguration="{\"Bottom\":[],\"Left\":[{\"id\":\"A\",\"label\":\"A\",\"type\":\"foundation.thermal.thermal\"}],\"Right\":[{\"id\":\"B\",\"label\":\"B\",\"type\":\"foundation.thermal.thermal\"}],\"Top\":[]}"
  Clock : Clock  Commented=on
  Compare To Constant : simulink/Logic and Bit Operations/Compare To Constant  Commented=on  relop=>=  const=295  OutDataTypeStr=boolean
  Constant : Constant  Commented=on  Value=1000000000
  Constant1 : Constant  Commented=on  Value=0
  Constant2 : Constant  Commented=on  Value=0
  From29 : From  Commented=on  GotoTag=A29
  From30 : From  Commented=on  GotoTag=A30
  From55 : From  Commented=on  GotoTag=T_1_6_RECEIVER
  From84 : From  Commented=on  GotoTag=T_INS
  Goto36 : Goto  Commented=on  GotoTag=A17
  Goto37 : Goto  Commented=on  GotoTag=A18
  Goto80 : Goto  Commented=on  GotoTag=T_INS
  Goto88 : Goto  Commented=on  GotoTag=A38
  Goto89 : Goto  Commented=on  GotoTag=A37_1
  Goto90 : Goto  Commented=on  GotoTag=A37_2
  Goto91 : Goto  Commented=on  GotoTag=A37_3
  HEATER_1 : Subsystem
      settings: PortSchema="{\"entries\":[{\"content\":{\"sides\":[{\"content\":{},\"type\":\"ConnectorPlacement.EquallySpacedRectSide\",\"uuid\":\"b560d365-df61-4763-a3d2-7aabc9c9e784\"},{\"content\":{\"side\":\"RIGHT\"},\"type\":\"ConnectorPlacement.EquallySpacedRectSide\",\"uuid\":\"d9aec98f-6504-4c51-a44b-0b1357bacb3d\"},{\"content\":{\"connectorIds\":[\"In1\"],\"side\":\"TOP\"},\"type\":\"ConnectorPlacement.EquallySpacedRectSide\",\"uuid\":\"3b51a013-3049-445c-99f3-fc99ed5dfc2c\"},{\"content\":{\"connectorIds\":[\"RConn1\"],\"side\":\"BOTTOM\"},\"type\":\"ConnectorPlacement.EquallySpacedRectSide\",\"uuid\":\"c2f75917-e2f0-4ab7-b39e-beaf9bfb560b\"}]},\"type\":\"ConnectorPlacement.EquallySpacedConnector\",\"uuid\":\"d6cdd11a-7162-4cf4-9c21-a4d4004f90d5\"}],\"packageUris\":[\"http://schema.mathworks.com/mf0/Connector/R2020b\"],\"version\":\"1.0\"}"
  HEATER_2 : Subsystem
      settings: PortSchema="{\"entries\":[{\"content\":{\"sides\":[{\"content\":{},\"type\":\"ConnectorPlacement.EquallySpacedRectSide\",\"uuid\":\"b560d365-df61-4763-a3d2-7aabc9c9e784\"},{\"content\":{\"side\":\"RIGHT\"},\"type\":\"ConnectorPlacement.EquallySpacedRectSide\",\"uuid\":\"d9aec98f-6504-4c51-a44b-0b1357bacb3d\"},{\"content\":{\"connectorIds\":[\"In1\"],\"side\":\"TOP\"},\"type\":\"ConnectorPlacement.EquallySpacedRectSide\",\"uuid\":\"3b51a013-3049-445c-99f3-fc99ed5dfc2c\"},{\"content\":{\"connectorIds\":[\"RConn1\"],\"side\":\"BOTTOM\"},\"type\":\"ConnectorPlacement.EquallySpacedRectSide\",\"uuid\":\"c2f75917-e2f0-4ab7-b39e-beaf9bfb560b\"}]},\"type\":\"ConnectorPlacement.EquallySpacedConnector\",\"uuid\":\"d6cdd11a-7162-4cf4-9c21-a4d4004f90d5\"}],\"packageUris\":[\"http://schema.mathworks.com/mf0/Connector/R2020b\"],\"version\":\"1.0\"}"
  HEATER_3 : Subsystem  Commented=on
      settings: PortSchema="{\"entries\":[{\"content\":{\"sides\":[{\"content\":{},\"type\":\"ConnectorPlacement.EquallySpacedRectSide\",\"uuid\":\"b560d365-df61-4763-a3d2-7aabc9c9e784\"},{\"content\":{\"side\":\"RIGHT\"},\"type\":\"ConnectorPlacement.EquallySpacedRectSide\",\"uuid\":\"d9aec98f-6504-4c51-a44b-0b1357bacb3d\"},{\"content\":{\"connectorIds\":[\"In1\"],\"side\":\"TOP\"},\"type\":\"ConnectorPlacement.EquallySpacedRectSide\",\"uuid\":\"3b51a013-3049-445c-99f3-fc99ed5dfc2c\"},{\"content\":{\"connectorIds\":[\"RConn1\"],\"side\":\"BOTTOM\"},\"type\":\"ConnectorPlacement.EquallySpacedRectSide\",\"uuid\":\"c2f75917-e2f0-4ab7-b39e-beaf9bfb560b\"}]},\"type\":\"ConnectorPlacement.EquallySpacedConnector\",\"uuid\":\"d6cdd11a-7162-4cf4-9c21-a4d4004f90d5\"}],\"packageUris\":[\"http://schema.mathworks.com/mf0/Connector/R2020b\"],\"version\":\"1.0\"}"
  HEATER_4 : Subsystem
      settings: PortSchema="{\"entries\":[{\"content\":{\"sides\":[{\"content\":{},\"type\":\"ConnectorPlacement.EquallySpacedRectSide\",\"uuid\":\"b560d365-df61-4763-a3d2-7aabc9c9e784\"},{\"content\":{\"side\":\"RIGHT\"},\"type\":\"ConnectorPlacement.EquallySpacedRectSide\",\"uuid\":\"d9aec98f-6504-4c51-a44b-0b1357bacb3d\"},{\"content\":{\"connectorIds\":[\"In1\"],\"side\":\"TOP\"},\"type\":\"ConnectorPlacement.EquallySpacedRectSide\",\"uuid\":\"3b51a013-3049-445c-99f3-fc99ed5dfc2c\"},{\"content\":{\"connectorIds\":[\"RConn1\"],\"side\":\"BOTTOM\"},\"type\":\"ConnectorPlacement.EquallySpacedRectSide\",\"uuid\":\"c2f75917-e2f0-4ab7-b39e-beaf9bfb560b\"}]},\"type\":\"ConnectorPlacement.EquallySpacedConnector\",\"uuid\":\"d6cdd11a-7162-4cf4-9c21-a4d4004f90d5\"}],\"packageUris\":[\"http://schema.mathworks.com/mf0/Connector/R2020b\"],\"version\":\"1.0\"}"
  HEATER_5 : Subsystem
      settings: PortSchema="{\"entries\":[{\"content\":{\"sides\":[{\"content\":{},\"type\":\"ConnectorPlacement.EquallySpacedRectSide\",\"uuid\":\"b560d365-df61-4763-a3d2-7aabc9c9e784\"},{\"content\":{\"side\":\"RIGHT\"},\"type\":\"ConnectorPlacement.EquallySpacedRectSide\",\"uuid\":\"d9aec98f-6504-4c51-a44b-0b1357bacb3d\"},{\"content\":{\"connectorIds\":[\"In1\"],\"side\":\"TOP\"},\"type\":\"ConnectorPlacement.EquallySpacedRectSide\",\"uuid\":\"3b51a013-3049-445c-99f3-fc99ed5dfc2c\"},{\"content\":{\"connectorIds\":[\"RConn1\"],\"side\":\"BOTTOM\"},\"type\":\"ConnectorPlacement.EquallySpacedRectSide\",\"uuid\":\"c2f75917-e2f0-4ab7-b39e-beaf9bfb560b\"}]},\"type\":\"ConnectorPlacement.EquallySpacedConnector\",\"uuid\":\"d6cdd11a-7162-4cf4-9c21-a4d4004f90d5\"}],\"packageUris\":[\"http://schema.mathworks.com/mf0/Connector/R2020b\"],\"version\":\"1.0\"}"
  HEATER_6 : Subsystem
      settings: PortSchema="{\"entries\":[{\"content\":{\"sides\":[{\"content\":{},\"type\":\"ConnectorPlacement.EquallySpacedRectSide\",\"uuid\":\"b560d365-df61-4763-a3d2-7aabc9c9e784\"},{\"content\":{\"side\":\"RIGHT\"},\"type\":\"ConnectorPlacement.EquallySpacedRectSide\",\"uuid\":\"d9aec98f-6504-4c51-a44b-0b1357bacb3d\"},{\"content\":{\"connectorIds\":[\"In1\"],\"side\":\"TOP\"},\"type\":\"ConnectorPlacement.EquallySpacedRectSide\",\"uuid\":\"3b51a013-3049-445c-99f3-fc99ed5dfc2c\"},{\"content\":{\"connectorIds\":[\"RConn1\"],\"side\":\"BOTTOM\"},\"type\":\"ConnectorPlacement.EquallySpacedRectSide\",\"uuid\":\"c2f75917-e2f0-4ab7-b39e-beaf9bfb560b\"}]},\"type\":\"ConnectorPlacement.EquallySpacedConnector\",\"uuid\":\"d6cdd11a-7162-4cf4-9c21-a4d4004f90d5\"}],\"packageUris\":[\"http://schema.mathworks.com/mf0/Connector/R2020b\"],\"version\":\"1.0\"}"
  HEATER_7 : Subsystem
      settings: PortSchema="{\"entries\":[{\"content\":{\"sides\":[{\"content\":{},\"type\":\"ConnectorPlacement.EquallySpacedRectSide\",\"uuid\":\"b560d365-df61-4763-a3d2-7aabc9c9e784\"},{\"content\":{\"side\":\"RIGHT\"},\"type\":\"ConnectorPlacement.EquallySpacedRectSide\",\"uuid\":\"d9aec98f-6504-4c51-a44b-0b1357bacb3d\"},{\"content\":{\"connectorIds\":[\"In1\"],\"side\":\"TOP\"},\"type\":\"ConnectorPlacement.EquallySpacedRectSide\",\"uuid\":\"3b51a013-3049-445c-99f3-fc99ed5dfc2c\"},{\"content\":{\"connectorIds\":[\"RConn1\"],\"side\":\"BOTTOM\"},\"type\":\"ConnectorPlacement.EquallySpacedRectSide\",\"uuid\":\"c2f75917-e2f0-4ab7-b39e-beaf9bfb560b\"}]},\"type\":\"ConnectorPlacement.EquallySpacedConnector\",\"uuid\":\"d6cdd11a-7162-4cf4-9c21-a4d4004f90d5\"}],\"packageUris\":[\"http://schema.mathworks.com/mf0/Connector/R2020b\"],\"version\":\"1.0\"}"
  HEATER_8 : Subsystem
      settings: PortSchema="{\"entries\":[{\"content\":{\"sides\":[{\"content\":{},\"type\":\"ConnectorPlacement.EquallySpacedRectSide\",\"uuid\":\"b560d365-df61-4763-a3d2-7aabc9c9e784\"},{\"content\":{\"side\":\"RIGHT\"},\"type\":\"ConnectorPlacement.EquallySpacedRectSide\",\"uuid\":\"d9aec98f-6504-4c51-a44b-0b1357bacb3d\"},{\"content\":{\"connectorIds\":[\"In1\"],\"side\":\"TOP\"},\"type\":\"ConnectorPlacement.EquallySpacedRectSide\",\"uuid\":\"3b51a013-3049-445c-99f3-fc99ed5dfc2c\"},{\"content\":{\"connectorIds\":[\"RConn1\"],\"side\":\"BOTTOM\"},\"type\":\"ConnectorPlacement.EquallySpacedRectSide\",\"uuid\":\"c2f75917-e2f0-4ab7-b39e-beaf9bfb560b\"}]},\"type\":\"ConnectorPlacement.EquallySpacedConnector\",\"uuid\":\"d6cdd11a-7162-4cf4-9c21-a4d4004f90d5\"}],\"packageUris\":[\"http://schema.mathworks.com/mf0/Connector/R2020b\"],\"version\":\"1.0\"}"
  Heat Flow Rate Sensor{1..43,46..58,87} (57 alike) : fl_lib/Thermal/Thermal Sensors/Heat Flow Rate Sensor
  Heat Flow Rate Sensor44 : fl_lib/Thermal/Thermal Sensors/Heat Flow Rate Sensor  Commented=on
  Heat Flow Rate Sensor45 : fl_lib/Thermal/Thermal Sensors/Heat Flow Rate Sensor  Commented=on
  LOAD_ALL : Scope  NumInputPorts=40
      settings: ActiveDisplayYMinimum=-23.14326  ActiveDisplayYMaximum=60.20368  DataLoggingVariableName=LOADS_ALL
  LOAD_ALL2 : Scope  NumInputPorts=26
      settings: ActiveDisplayYMinimum=-1.12539  ActiveDisplayYMaximum=9.98538
  L_A{1..16,19..28,31..34,36,38} (32 alike) : nesl_utility/PS-Simulink Converter  PhysicalDomain=network_engine_domain  SubClassName=ps_output  LeftPortType=input  RightPortType=output  PseudoPeriodic=off  Frequencies=[]  VectorFormat=inherit  Unit=inherit  AffineConversion=off
  L_A17 : nesl_utility/PS-Simulink Converter  Commented=on  PhysicalDomain=network_engine_domain  SubClassName=ps_output  LeftPortType=input  RightPortType=output  PseudoPeriodic=off  Frequencies=[]  VectorFormat=inherit  Unit=inherit  AffineConversion=off
  L_A18 : nesl_utility/PS-Simulink Converter  Commented=on  PhysicalDomain=network_engine_domain  SubClassName=ps_output  LeftPortType=input  RightPortType=output  PseudoPeriodic=off  Frequencies=[]  VectorFormat=inherit  Unit=inherit  AffineConversion=off
  L_A29 : nesl_utility/PS-Simulink Converter  Commented=on  PhysicalDomain=network_engine_domain  SubClassName=ps_output  LeftPortType=input  RightPortType=output  PseudoPeriodic=off  Frequencies=[]  VectorFormat=inherit  Unit=inherit  AffineConversion=off
  L_A37.1 : nesl_utility/PS-Simulink Converter  PhysicalDomain=network_engine_domain  SubClassName=ps_output  LeftPortType=input  RightPortType=output  PseudoPeriodic=off  Frequencies=[]  VectorFormat=inherit  Unit=inherit  AffineConversion=off
  L_A37.2 : nesl_utility/PS-Simulink Converter  PhysicalDomain=network_engine_domain  SubClassName=ps_output  LeftPortType=input  RightPortType=output  PseudoPeriodic=off  Frequencies=[]  VectorFormat=inherit  Unit=inherit  AffineConversion=off
  L_A37.3 : nesl_utility/PS-Simulink Converter  PhysicalDomain=network_engine_domain  SubClassName=ps_output  LeftPortType=input  RightPortType=output  PseudoPeriodic=off  Frequencies=[]  VectorFormat=inherit  Unit=inherit  AffineConversion=off
  L_A37.4 : nesl_utility/PS-Simulink Converter  Commented=on  PhysicalDomain=network_engine_domain  SubClassName=ps_output  LeftPortType=input  RightPortType=output  PseudoPeriodic=off  Frequencies=[]  VectorFormat=inherit  Unit=inherit  AffineConversion=off
  L_A37.5 : nesl_utility/PS-Simulink Converter  Commented=on  PhysicalDomain=network_engine_domain  SubClassName=ps_output  LeftPortType=input  RightPortType=output  PseudoPeriodic=off  Frequencies=[]  VectorFormat=inherit  Unit=inherit  AffineConversion=off
  L_A37.6 : nesl_utility/PS-Simulink Converter  Commented=on  PhysicalDomain=network_engine_domain  SubClassName=ps_output  LeftPortType=input  RightPortType=output  PseudoPeriodic=off  Frequencies=[]  VectorFormat=inherit  Unit=inherit  AffineConversion=off
  L_B{1..9,13..23,25..27} (23 alike) : nesl_utility/PS-Simulink Converter  PhysicalDomain=network_engine_domain  SubClassName=ps_output  LeftPortType=input  RightPortType=output  PseudoPeriodic=off  Frequencies=[]  VectorFormat=inherit  Unit=inherit  AffineConversion=off
  L_B10.1 : nesl_utility/PS-Simulink Converter  PhysicalDomain=network_engine_domain  SubClassName=ps_output  LeftPortType=input  RightPortType=output  PseudoPeriodic=off  Frequencies=[]  VectorFormat=inherit  Unit=inherit  AffineConversion=off
  L_B10.2 : nesl_utility/PS-Simulink Converter  PhysicalDomain=network_engine_domain  SubClassName=ps_output  LeftPortType=input  RightPortType=output  PseudoPeriodic=off  Frequencies=[]  VectorFormat=inherit  Unit=inherit  AffineConversion=off
  L_B10.3 : nesl_utility/PS-Simulink Converter  PhysicalDomain=network_engine_domain  SubClassName=ps_output  LeftPortType=input  RightPortType=output  PseudoPeriodic=off  Frequencies=[]  VectorFormat=inherit  Unit=inherit  AffineConversion=off
  Logical Operator : Logic  Commented=on  Operator=OR  AllPortsSameDT=off
  Memory : Memory  Commented=on  LinearizeMemory=on  LinearizeAsDelay=on
  R_A1 : Lookup_n-D  NumberOfTableDimensions=1  BreakpointsForDimension1=xt  Table=res_A1  InternalRulePriority=Speed  RndMeth=Simplest
  R_A10 : Lookup_n-D  NumberOfTableDimensions=1  BreakpointsForDimension1=xt  Table=res_A10  InternalRulePriority=Speed  RndMeth=Simplest
  R_A12 : Lookup_n-D  NumberOfTableDimensions=1  BreakpointsForDimension1=xt  Table=res_A12  InternalRulePriority=Speed  RndMeth=Simplest
  R_A14 : Lookup_n-D  NumberOfTableDimensions=1  BreakpointsForDimension1=xt  Table=res_A14  InternalRulePriority=Speed  RndMeth=Simplest
  R_A15 : Lookup_n-D  NumberOfTableDimensions=1  BreakpointsForDimension1=xt  Table=res_A15  InternalRulePriority=Speed  RndMeth=Simplest
  R_A2 : Lookup_n-D  NumberOfTableDimensions=1  BreakpointsForDimension1=xt  Table=res_A38  InternalRulePriority=Speed  RndMeth=Simplest
  R_A20 : Lookup_n-D  NumberOfTableDimensions=1  BreakpointsForDimension1=xt  Table=res_A20  InternalRulePriority=Speed  RndMeth=Simplest
  R_A21 : Lookup_n-D  NumberOfTableDimensions=1  BreakpointsForDimension1=xt  Table=res_A21  InternalRulePriority=Speed  RndMeth=Simplest
  R_A24 : Lookup_n-D  NumberOfTableDimensions=1  BreakpointsForDimension1=xt  Table=res_A24  InternalRulePriority=Speed  RndMeth=Simplest
  R_A25 : Lookup_n-D  NumberOfTableDimensions=1  BreakpointsForDimension1=xt  Table=res_A25  InternalRulePriority=Speed  RndMeth=Simplest
  R_A28 : Lookup_n-D  NumberOfTableDimensions=1  BreakpointsForDimension1=xt  Table=res_A28  InternalRulePriority=Speed  RndMeth=Simplest
  R_A37.{1..6} (6 alike) : Lookup_n-D  NumberOfTableDimensions=1  BreakpointsForDimension1=xt  Table=res_A37  InternalRulePriority=Speed  RndMeth=Simplest
  R_A38 : Lookup_n-D  NumberOfTableDimensions=1  BreakpointsForDimension1=xt  Table=res_A38  InternalRulePriority=Speed  RndMeth=Simplest
  R_A4 : Lookup_n-D  NumberOfTableDimensions=1  BreakpointsForDimension1=xt  Table=res_A2  InternalRulePriority=Speed  RndMeth=Simplest
  R_A5 : Lookup_n-D  NumberOfTableDimensions=1  BreakpointsForDimension1=xt  Table=res_A5  InternalRulePriority=Speed  RndMeth=Simplest
  R_A8 : Lookup_n-D  NumberOfTableDimensions=1  BreakpointsForDimension1=xt  Table=res_A8  InternalRulePriority=Speed  RndMeth=Simplest
  R_A9 : Lookup_n-D  NumberOfTableDimensions=1  BreakpointsForDimension1=xt  Table=res_A9  InternalRulePriority=Speed  RndMeth=Simplest
  SAMPLE_CONN : fl_lib/Thermal/Thermal Elements/Variable Thermal Resistance  Commented=on  R_min=0 K/W  T_specify=off  T_priority=None  T=0 K  T_nominal_specify=off  T_nominal_value=1  T_nominal_unit=K  Q_specify=off  Q_priority=None  Q=0 W  Q_nominal_specify=off  Q_nominal_value=1  Q_nominal_unit=W
      settings: InternalSimscapePortConfiguration="{\"Bottom\":[],\"Left\":[{\"id\":\"A\",\"label\":\"A\",\"type\":\"foundation.thermal.thermal\"},{\"id\":\"R\",\"label\":\"R\",\"type\":\"input\"}],\"Right\":[{\"id\":\"B\",\"label\":\"B\",\"type\":\"foundation.thermal.thermal\"}],\"Top\":[]}"
  STAGE_ROTARY : nesl_utility/PS-Simulink Converter  PhysicalDomain=network_engine_domain  SubClassName=ps_output  LeftPortType=input  RightPortType=output  PseudoPeriodic=off  Frequencies=[]  VectorFormat=inherit  Unit=inherit  AffineConversion=off
  Simulink-PS Converter : nesl_utility/Simulink-PS Converter  Commented=on  PhysicalDomain=network_engine_domain  SubClassName=ps_input  LeftPortType=input  RightPortType=output  PseudoPeriodic=off  Frequencies=[]  NoiseDistribution=none  NoiseParameters=[]  Unit=1  AffineConversion=off  FilteringAndDerivatives=provide  SimscapeFilterOrder=1  InputFilterTimeConstant=0.001  UdotUserProvided=0
  Simulink-PS Converter{1..22} (22 alike) : nesl_utility/Simulink-PS Converter  PhysicalDomain=network_engine_domain  SubClassName=ps_input  LeftPortType=input  RightPortType=output  PseudoPeriodic=off  Frequencies=[]  NoiseDistribution=none  NoiseParameters=[]  Unit=1  AffineConversion=off  FilteringAndDerivatives=provide  SimscapeFilterOrder=1  InputFilterTimeConstant=0.001  UdotUserProvided=0
  Solver Configuration : nesl_utility/Solver Configuration  PhysicalDomain=network_engine_domain  SubClassName=solver  LeftPortType=input  RightPortType=generic  Tones=[]  Harmonics=[]  SimulateNoise=off  Profile=off  UseLocalSampling=off  EnableSwitchedLinearOptims=on  FrequencyDomain=off  UseCCode=off  RelTol=0.001  AbsTol=0.001  MinStep=1e-09  ToWorkspace=off  RevertToSquareIcSolve=off  NumHomotopyIterations=100  PhasorMode=off  PhasorModeNumHarmonics=1  ConsistencySolver=NEWTON_FTOL  IndexReductionMethod=DerivativeReplacement  DoDC=off  ResidualTolerance=1e-09  ConsistencyTolSource=GLOBAL  ConsistencyAbsTol=0.001  ConsistencyRelTol=0.001  ConsistencyTolFactor=0.001  UseLocalSolver=off  LocalSolverChoice=NE_BACKWARD_EULER_ADVANCER  ResolveIndetEquations=on  FunctionEvalNumThread=1  LocalSolverSampleTime=0.001  DoFixedCost=off  MaxNonlinIter=3  MaxModeIter=2  ComputeImpulses=off  ImpulseIterations=2  LinearAlgebra=auto  LinearAlgebraNumThread=0  EquationFormulation=NE_TIME_EF  DelaysMemoryBudget=1024  AutomaticFiltering=on  FilteringTimeConstant=0.001  PartitionStorageMethod=AS_NEEDED  PartitionMemoryBudget=1024  PartitionMethod=ROBUST  MultibodyUseLocalSolver=off  MultibodyLocalSolverChoice=ODE1  MultibodyLocalSolverSampleTime=0.001
  Subsystem : Subsystem
  Switch : Switch  Commented=on  Threshold=295.15  ZeroCross=off  SaturateOnIntegerOverflow=off  InputSameDT=off
  Switch1 : Switch  Commented=on  Criteria=u2 > Threshold  Threshold=48000  ZeroCross=off  SaturateOnIntegerOverflow=off  InputSameDT=off
  TEMP_AUX_COMPONENTS1 : Scope  NumInputPorts=12
      settings: ActiveDisplayYMinimum=3.45129  ActiveDisplayYMaximum=333.05382
  TEMP_COLD_STAGE : Scope  NumInputPorts=11
      settings: ActiveDisplayYMinimum=-36.89695033266419  ActiveDisplayYMaximum=332.07255299397775  DataLoggingVariableName=TEMP_COLD_STAGE
  TEMP_HOT_STAGE : Scope  NumInputPorts=11
      settings: ActiveDisplayYMinimum=-30.5354  ActiveDisplayYMaximum=331.3393
  TEMP_MOTION_STAGES : Scope
      settings: ActiveDisplayYMinimum=291.83189  ActiveDisplayYMaximum=325.01302  DataLoggingVariableName=ScopeData4
  T_1.2_BRAID_END : nesl_utility/PS-Simulink Converter  PhysicalDomain=network_engine_domain  SubClassName=ps_output  LeftPortType=input  RightPortType=output  PseudoPeriodic=off  Frequencies=[]  VectorFormat=inherit  Unit=inherit  AffineConversion=off
  T_1.2_BRAID_START : nesl_utility/PS-Simulink Converter  PhysicalDomain=network_engine_domain  SubClassName=ps_output  LeftPortType=input  RightPortType=output  PseudoPeriodic=off  Frequencies=[]  VectorFormat=inherit  Unit=inherit  AffineConversion=off
  T_1.3_BUSBAR : nesl_utility/PS-Simulink Converter  PhysicalDomain=network_engine_domain  SubClassName=ps_output  LeftPortType=input  RightPortType=output  PseudoPeriodic=off  Frequencies=[]  VectorFormat=inherit  Unit=inherit  AffineConversion=off
  T_1.4_BRAID_END : nesl_utility/PS-Simulink Converter  PhysicalDomain=network_engine_domain  SubClassName=ps_output  LeftPortType=input  RightPortType=output  PseudoPeriodic=off  Frequencies=[]  VectorFormat=inherit  Unit=inherit  AffineConversion=off
  T_1.4_BRAID_START : nesl_utility/PS-Simulink Converter  PhysicalDomain=network_engine_domain  SubClassName=ps_output  LeftPortType=input  RightPortType=output  PseudoPeriodic=off  Frequencies=[]  VectorFormat=inherit  Unit=inherit  AffineConversion=off
  T_1.5_PULLEY : nesl_utility/PS-Simulink Converter  PhysicalDomain=network_engine_domain  SubClassName=ps_output  LeftPortType=input  RightPortType=output  PseudoPeriodic=off  Frequencies=[]  VectorFormat=inherit  Unit=inherit  AffineConversion=off
  T_1.6_RECEIVER : nesl_utility/PS-Simulink Converter  PhysicalDomain=network_engine_domain  SubClassName=ps_output  LeftPortType=input  RightPortType=output  PseudoPeriodic=off  Frequencies=[]  VectorFormat=inherit  Unit=inherit  AffineConversion=off
  T_1.7_SAMPLE_HOLDER : nesl_utility/PS-Simulink Converter  PhysicalDomain=network_engine_domain  SubClassName=ps_output  LeftPortType=input  RightPortType=output  PseudoPeriodic=off  Frequencies=[]  VectorFormat=inherit  Unit=inherit  AffineConversion=off
  T_1.8_SAMPLE : nesl_utility/PS-Simulink Converter  PhysicalDomain=network_engine_domain  SubClassName=ps_output  LeftPortType=input  RightPortType=output  PseudoPeriodic=off  Frequencies=[]  VectorFormat=inherit  Unit=inherit  AffineConversion=off
  T_2.2_SHIELD : nesl_utility/PS-Simulink Converter  PhysicalDomain=network_engine_domain  SubClassName=ps_output  LeftPortType=input  RightPortType=output  PseudoPeriodic=off  Frequencies=[]  VectorFormat=inherit  Unit=inherit  AffineConversion=off
  T_2.3.1_BRAID : nesl_utility/PS-Simulink Converter  PhysicalDomain=network_engine_domain  SubClassName=ps_output  LeftPortType=input  RightPortType=output  PseudoPeriodic=off  Frequencies=[]  VectorFormat=inherit  Unit=inherit  AffineConversion=off
  T_2.3.3_BRAID : nesl_utility/PS-Simulink Converter  PhysicalDomain=network_engine_domain  SubClassName=ps_output  LeftPortType=input  RightPortType=output  PseudoPeriodic=off  Frequencies=[]  VectorFormat=inherit  Unit=inherit  AffineConversion=off
  T_2.4.1_SHIELD : nesl_utility/PS-Simulink Converter  PhysicalDomain=network_engine_domain  SubClassName=ps_output  LeftPortType=input  RightPortType=output  PseudoPeriodic=off  Frequencies=[]  VectorFormat=inherit  Unit=inherit  AffineConversion=off
  T_2.4.2_SHIELD : nesl_utility/PS-Simulink Converter  PhysicalDomain=network_engine_domain  SubClassName=ps_output  LeftPortType=input  RightPortType=output  PseudoPeriodic=off  Frequencies=[]  VectorFormat=inherit  Unit=inherit  AffineConversion=off
  T_2.4.3_SHIELD : nesl_utility/PS-Simulink Converter  PhysicalDomain=network_engine_domain  SubClassName=ps_output  LeftPortType=input  RightPortType=output  PseudoPeriodic=off  Frequencies=[]  VectorFormat=inherit  Unit=inherit  AffineConversion=off
  T_2.5.1_BRAID : nesl_utility/PS-Simulink Converter  PhysicalDomain=network_engine_domain  SubClassName=ps_output  LeftPortType=input  RightPortType=output  PseudoPeriodic=off  Frequencies=[]  VectorFormat=inherit  Unit=inherit  AffineConversion=off
  T_2.5.3_BRAID : nesl_utility/PS-Simulink Converter  PhysicalDomain=network_engine_domain  SubClassName=ps_output  LeftPortType=input  RightPortType=output  PseudoPeriodic=off  Frequencies=[]  VectorFormat=inherit  Unit=inherit  AffineConversion=off
  T_2.6_SHIELD : nesl_utility/PS-Simulink Converter  PhysicalDomain=network_engine_domain  SubClassName=ps_output  LeftPortType=input  RightPortType=output  PseudoPeriodic=off  Frequencies=[]  VectorFormat=inherit  Unit=inherit  AffineConversion=off
  T_4.7.{1..6,12,45,56,234} (10 alike) : nesl_utility/PS-Simulink Converter  PhysicalDomain=network_engine_domain  SubClassName=ps_output  LeftPortType=input  RightPortType=output  PseudoPeriodic=off  Frequencies=[]  VectorFormat=inherit  Unit=inherit  AffineConversion=off
  T_4.7.1X : nesl_utility/PS-Simulink Converter  PhysicalDomain=network_engine_domain  SubClassName=ps_output  LeftPortType=input  RightPortType=output  PseudoPeriodic=off  Frequencies=[]  VectorFormat=inherit  Unit=inherit  AffineConversion=off
  T_4.7.6X : nesl_utility/PS-Simulink Converter  PhysicalDomain=network_engine_domain  SubClassName=ps_output  LeftPortType=input  RightPortType=output  PseudoPeriodic=off  Frequencies=[]  VectorFormat=inherit  Unit=inherit  AffineConversion=off
  T_A{1..2,4..5,8..10,12,14..15,20..21,24..25,28,38} (16 alike) : nesl_utility/PS-Simulink Converter  PhysicalDomain=network_engine_domain  SubClassName=ps_output  LeftPortType=input  RightPortType=output  PseudoPeriodic=off  Frequencies=[]  VectorFormat=inherit  Unit=inherit  AffineConversion=off
  T_A37.{1..6} (6 alike) : nesl_utility/PS-Simulink Converter  PhysicalDomain=network_engine_domain  SubClassName=ps_output  LeftPortType=input  RightPortType=output  PseudoPeriodic=off  Frequencies=[]  VectorFormat=inherit  Unit=inherit  AffineConversion=off
  T_COLD_HEAD : nesl_utility/PS-Simulink Converter  PhysicalDomain=network_engine_domain  SubClassName=ps_output  LeftPortType=input  RightPortType=output  PseudoPeriodic=off  Frequencies=[]  VectorFormat=inherit  Unit=inherit  AffineConversion=off
  T_HOT_HEAD : nesl_utility/PS-Simulink Converter  PhysicalDomain=network_engine_domain  SubClassName=ps_output  LeftPortType=input  RightPortType=output  PseudoPeriodic=off  Frequencies=[]  VectorFormat=inherit  Unit=inherit  AffineConversion=off
  T_INS : nesl_utility/PS-Simulink Converter  Commented=on  PhysicalDomain=network_engine_domain  SubClassName=ps_output  LeftPortType=input  RightPortType=output  PseudoPeriodic=off  Frequencies=[]  VectorFormat=inherit  Unit=inherit  AffineConversion=off
  Temperature Sensor{1..41} (41 alike) : fl_lib/Thermal/Thermal Sensors/Temperature Sensor  temperature_measure=foundation.enum.MeasurementReference.difference
  Temperature Source : fl_lib/Thermal/Thermal Sources/Temperature Source  Commented=on  temperature=4.2 K
  Temperature Source{1..15} (15 alike) : fl_lib/Thermal/Thermal Sources/Temperature Source  temperature=Temp_Environment K
  Thermal Reference{1..41} (41 alike) : fl_lib/Thermal/Thermal Elements/Thermal Reference
  W_COLD_HEAD : nesl_utility/PS-Simulink Converter  PhysicalDomain=network_engine_domain  SubClassName=ps_output  LeftPortType=input  RightPortType=output  PseudoPeriodic=off  Frequencies=[]  VectorFormat=inherit  Unit=inherit  AffineConversion=off
  W_HOT_HEAD : nesl_utility/PS-Simulink Converter  PhysicalDomain=network_engine_domain  SubClassName=ps_output  LeftPortType=input  RightPortType=output  PseudoPeriodic=off  Frequencies=[]  VectorFormat=inherit  Unit=inherit  AffineConversion=off
  wires:
  STAGE_ROTARY/1 -> [SM_ROTARY_TEMP]
  T_A1/1 -> R_A1/1
  R_A1/1 -> Simulink-PS Converter2/1
  T_A5/1 -> R_A5/1
  R_A5/1 -> Simulink-PS Converter3/1
  R_A8/1 -> Simulink-PS Converter4/1
  T_A8/1 -> R_A8/1
  R_A10/1 -> Simulink-PS Converter12/1
  T_A10/1 -> R_A10/1
  T_A9/1 -> R_A9/1
  R_A9/1 -> Simulink-PS Converter13/1
  [A1] -> LOAD_ALL/1
  [A8] -> LOAD_ALL/8
  [A11] -> LOAD_ALL/11
  [A10] -> LOAD_ALL/10
  [A7] -> LOAD_ALL/7
  [A9] -> LOAD_ALL/9
  [A12] -> LOAD_ALL/12
  [A21] -> LOAD_ALL/21
  [A14] -> LOAD_ALL/14
  [A19] -> LOAD_ALL/19
  [A18] -> LOAD_ALL/18
  [A13] -> LOAD_ALL/13
  [A20] -> LOAD_ALL/20
  [A16] -> LOAD_ALL/16
  [A17] -> LOAD_ALL/17
  [A15] -> LOAD_ALL/15
  [A35] -> LOAD_ALL/35
  [A36] -> LOAD_ALL/36
  From30/1 -> LOAD_ALL/30
  From29/1 -> LOAD_ALL/29
  [A25] -> LOAD_ALL/25
  [A34] -> LOAD_ALL/34
  [A2] -> LOAD_ALL/2
  [A3] -> LOAD_ALL/3
  L_A5/1 -> [A5]
  L_A1/1 -> [A1]
  [A4] -> LOAD_ALL/4
  [A5] -> LOAD_ALL/5
  [A6] -> LOAD_ALL/6
  L_A6/1 -> [A6]
  L_A7/1 -> [A7]
  L_A8/1 -> [A8]
  L_A9/1 -> [A9]
  L_A10/1 -> [A10]
  L_A11/1 -> [A11]
  [A26] -> LOAD_ALL/26
  L_A18/1 -> Goto37/1
  L_A19/1 -> [A19]
  [A33] -> LOAD_ALL/33
  [A32] -> LOAD_ALL/32
  [A31] -> LOAD_ALL/31
  L_B3/1 -> [B3]
  L_B4/1 -> [B4]
  L_B23/1 -> [B23]
  L_B22/1 -> [B22]
  Constant/1 -> Switch/3
  Switch/1 -> Simulink-PS Converter/1
  Constant1/1 -> Switch/1
  [T_1_8_SAMPLE] -> TEMP_COLD_STAGE/11
  T_1.8_SAMPLE/1 -> [T_1_8_SAMPLE]
  T_1.6_RECEIVER/1 -> [T_1_6_RECEIVER]
  [T_1_6_RECEIVER] -> TEMP_COLD_STAGE/9
  [T_1_6_RECEIVER] -> HEATER_1/1(In1)
  [T_1_2_BRAID_START] -> TEMP_COLD_STAGE/3
  [T_4_7_1] -> HEATER_2/1(In1)
  T_1.7_SAMPLE_HOLDER/1 -> [T_1_7_HOLDER]
  [T_1_7_HOLDER] -> TEMP_COLD_STAGE/10
  T_1.4_BRAID_END/1 -> [T_1_4_BRAID_END]
  T_1.4_BRAID_START/1 -> [T_1_4_BRAID_START]
  T_1.3_BUSBAR/1 -> [T_1_3_BUSBAR]
  [T_1_4_BRAID_END] -> TEMP_COLD_STAGE/7
  [T_1_4_BRAID_START] -> TEMP_COLD_STAGE/6
  [T_1_3_BUSBAR] -> TEMP_COLD_STAGE/5
  [T_1_2_BRAID_END] -> TEMP_COLD_STAGE/4
  T_1.5_PULLEY/1 -> [T_1_5_PULLEY]
  [T_1_5_PULLEY] -> TEMP_COLD_STAGE/8
  R_A4/1 -> Simulink-PS Converter11/1
  T_A4/1 -> R_A4/1
  L_A4/1 -> [A4]
  T_1.2_BRAID_END/1 -> [T_1_2_BRAID_END]
  L_B16/1 -> [B16]
  T_A28/1 -> R_A28/1
  R_A28/1 -> Simulink-PS Converter7/1
  L_A28/1 -> [A28]
  L_A25/1 -> [A25]
  R_A25/1 -> Simulink-PS Converter8/1
  T_A25/1 -> R_A25/1
  T_A24/1 -> R_A24/1
  R_A24/1 -> Simulink-PS Converter14/1
  L_A24/1 -> [A24]
  L_A33/1 -> [A33]
  L_B19/1 -> [B19]
  L_B20/1 -> [B20]
  L_B2/1 -> [B2]
  L_A32/1 -> [A32]
  L_A31/1 -> [A31]
  L_B13/1 -> [B13]
  L_B15/1 -> [B15]
  L_B14/1 -> [B14]
  R_A21/1 -> Simulink-PS Converter15/1
  T_A21/1 -> R_A21/1
  L_A21/1 -> [A21]
  L_A20/1 -> [A20]
  R_A20/1 -> Simulink-PS Converter16/1
  T_A20/1 -> R_A20/1
  L_B18/1 -> [B18]
  L_B17/1 -> [B17]
  L_A17/1 -> Goto36/1
  L_B1/1 -> [B1]
  L_A2/1 -> [A2]
  L_A3/1 -> [A3]
  [A22] -> LOAD_ALL/22
  [A23] -> LOAD_ALL/23
  [A24] -> LOAD_ALL/24
  [A27] -> LOAD_ALL/27
  [A28] -> LOAD_ALL/28
  L_A34/1 -> [A34]
  [B23] -> LOAD_ALL2/23
  [B8] -> LOAD_ALL2/8
  [B20] -> LOAD_ALL2/20
  [B10_2] -> LOAD_ALL2/11
  [B21] -> LOAD_ALL2/21
  [B6] -> LOAD_ALL2/6
  [B4] -> LOAD_ALL2/4
  [B5] -> LOAD_ALL2/5
  [B2] -> LOAD_ALL2/2
  [B13] -> LOAD_ALL2/13
  [B14] -> LOAD_ALL2/14
  [B22] -> LOAD_ALL2/22
  [B10_1] -> LOAD_ALL2/10
  [B7] -> LOAD_ALL2/7
  [B1] -> LOAD_ALL2/1
  [B17] -> LOAD_ALL2/17
  [B25] -> LOAD_ALL2/24
  [B10_3] -> LOAD_ALL2/12
  [B16] -> LOAD_ALL2/16
  [B15] -> LOAD_ALL2/15
  [B18] -> LOAD_ALL2/18
  [B19] -> LOAD_ALL2/19
  [B9] -> LOAD_ALL2/9
  [B3] -> LOAD_ALL2/3
  L_B21/1 -> [B21]
  T_1.2_BRAID_START/1 -> [T_1_2_BRAID_START]
  [SM_ROTARY_TEMP] -> TEMP_MOTION_STAGES/1
  [W_COLD_HEAD] -> TEMP_COLD_STAGE/1
  [T_COLD_HEAD] -> TEMP_COLD_STAGE/2
  T_COLD_HEAD/1 -> [T_COLD_HEAD]
  W_COLD_HEAD/1 -> [W_COLD_HEAD]
  Constant2/1 -> Switch1/3
  From55/1 -> Switch1/1
  Clock/1 -> Switch1/2
  Compare To Constant/1 -> Logical Operator/2
  Switch1/1 -> Compare To Constant/1
  Memory/1 -> Logical Operator/1
  Logical Operator/1 -> Memory/1, Switch/2
  T_2.2_SHIELD/1 -> [T_2_2_SHIELD]
  T_2.3.1_BRAID/1 -> [T_2_3_1_BRAID]
  T_2.3.3_BRAID/1 -> [T_2_3_3_BRAID]
  T_2.4.3_SHIELD/1 -> [T_2_4_3_SHIELD]
  T_2.4.2_SHIELD/1 -> [T_2_4_2_SHIELD]
  T_2.4.1_SHIELD/1 -> [T_2_4_1_SHIELD]
  T_2.5.1_BRAID/1 -> [T_2_5_1_BRAID]
  T_2.5.3_BRAID/1 -> [T_2_5_3_BRAID]
  T_2.6_SHIELD/1 -> [T_2_6_SHIELD]
  [T_HOT_HEAD] -> TEMP_HOT_STAGE/2
  [W_HOT_HEAD] -> TEMP_HOT_STAGE/1
  [T_2_5_1_BRAID] -> TEMP_HOT_STAGE/9
  [T_2_2_SHIELD] -> TEMP_HOT_STAGE/3
  [T_2_3_1_BRAID] -> TEMP_HOT_STAGE/4
  [T_2_6_SHIELD] -> TEMP_HOT_STAGE/11
  [T_2_3_3_BRAID] -> TEMP_HOT_STAGE/5
  [T_2_4_1_SHIELD] -> TEMP_HOT_STAGE/6
  [T_2_5_3_BRAID] -> TEMP_HOT_STAGE/10
  [T_2_4_3_SHIELD] -> TEMP_HOT_STAGE/8
  [T_2_4_2_SHIELD] -> TEMP_HOT_STAGE/7
  W_HOT_HEAD/1 -> [W_HOT_HEAD]
  T_HOT_HEAD/1 -> [T_HOT_HEAD]
  [T_1_4_BRAID_END] -> HEATER_4/1(In1)
  [T_1_3_BUSBAR] -> HEATER_5/1(In1)
  [T_1_2_BRAID_END] -> HEATER_6/1(In1)
  [T_2_3_3_BRAID] -> HEATER_7/1(In1)
  [T_2_4_2_SHIELD] -> HEATER_8/1(In1)
  T_A37.1/1 -> R_A37.1/1
  R_A37.1/1 -> Simulink-PS Converter1/1
  R_A37.2/1 -> Simulink-PS Converter5/1
  T_A37.2/1 -> R_A37.2/1
  R_A37.3/1 -> Simulink-PS Converter6/1
  T_A37.3/1 -> R_A37.3/1
  T_A15/1 -> R_A15/1
  R_A15/1 -> Simulink-PS Converter9/1
  T_A14/1 -> R_A14/1
  R_A14/1 -> Simulink-PS Converter10/1
  T_A12/1 -> R_A12/1
  R_A12/1 -> Simulink-PS Converter17/1
  T_A38/1 -> R_A38/1
  R_A38/1 -> Simulink-PS Converter18/1
  L_B25/1 -> [B25]
  L_B10.1/1 -> [B10_1]
  L_B10.3/1 -> [B10_3]
  L_B10.2/1 -> [B10_2]
  L_A37.1/1 -> [A37_1]
  L_A37.2/1 -> [A37_2]
  L_A37.3/1 -> [A37_3]
  L_B8/1 -> [B8]
  L_B7/1 -> [B7]
  L_A16/1 -> [A16]
  L_A13/1 -> [A13]
  L_A12/1 -> [A12]
  L_B9/1 -> [B9]
  L_A14/1 -> [A14]
  L_A15/1 -> [A15]
  L_A36/1 -> [A36]
  L_A38/1 -> [A38]
  L_A26/1 -> [A26]
  L_A27/1 -> [A27]
  [A37_2] -> LOAD_ALL/38
  [A37_1] -> LOAD_ALL/37
  [A38] -> LOAD_ALL/40
  [A37_3] -> LOAD_ALL/39
  L_A23/1 -> [A23]
  L_A22/1 -> [A22]
  L_B5/1 -> [B5]
  L_B6/1 -> [B6]
  T_4.7.1X/1 -> TEMP_AUX_COMPONENTS1/12
  T_4.7.1/1 -> [T_4_7_1], TEMP_AUX_COMPONENTS1/11
  T_4.7.12/1 -> TEMP_AUX_COMPONENTS1/10
  T_4.7.2/1 -> TEMP_AUX_COMPONENTS1/9
  T_4.7.234/1 -> TEMP_AUX_COMPONENTS1/8
  T_4.7.3/1 -> TEMP_AUX_COMPONENTS1/7
  T_4.7.4/1 -> TEMP_AUX_COMPONENTS1/6
  T_4.7.45/1 -> TEMP_AUX_COMPONENTS1/5
  T_4.7.5/1 -> TEMP_AUX_COMPONENTS1/4
  T_4.7.56/1 -> TEMP_AUX_COMPONENTS1/3
  T_4.7.6/1 -> TEMP_AUX_COMPONENTS1/2
  T_4.7.6X/1 -> TEMP_AUX_COMPONENTS1/1
  T_INS/1 -> Goto80/1
  From84/1 -> HEATER_3/1(In1)
  L_B26/1 -> [B26]
  [B26] -> LOAD_ALL2/25
  L_B27/1 -> [B27]
  [B27] -> LOAD_ALL2/26
  L_A29/1 -> Goto88/1
  T_A2/1 -> R_A2/1
  R_A2/1 -> Simulink-PS Converter19/1
  L_A37.6/1 -> Goto91/1
  L_A37.4/1 -> Goto89/1
  L_A37.5/1 -> Goto90/1
  T_A37.5/1 -> R_A37.5/1
  R_A37.5/1 -> Simulink-PS Converter21/1
  R_A37.6/1 -> Simulink-PS Converter22/1
  T_A37.6/1 -> R_A37.6/1
  R_A37.4/1 -> Simulink-PS Converter20/1
  T_A37.4/1 -> R_A37.4/1
  connections:
  Thermal Reference7/LConn1 -- Temperature Sensor6/RConn1
  Temperature Sensor6/RConn2 -- T_1.6_RECEIVER/LConn1
  Temperature Sensor6/LConn1 -- 1.6_SAMPLE_RECEIVER/LConn3
  B3/RConn1 -- Temperature Source1/LConn1
  HEATER_1/RConn1 -- 1.6_SAMPLE_RECEIVER/LConn2
  Heat Flow Rate Sensor30/RConn2 -- A10/RConn1
  A11/LConn1 -- 1.7_SAMPLE_HOLDER/RConn1
  Temperature Sensor1/LConn1 -- 1.8_SAMPLE/LConn2
  Thermal Reference1/LConn1 -- Temperature Sensor1/RConn1
  T_1.8_SAMPLE/LConn1 -- Temperature Sensor1/RConn2
  Thermal Reference2/LConn1 -- Temperature Sensor2/RConn1
  Temperature Sensor2/RConn2 -- T_1.7_SAMPLE_HOLDER/LConn1
  Temperature Sensor2/LConn1 -- 1.7_SAMPLE_HOLDER/LConn2
  Thermal Reference6/LConn1 -- Temperature Sensor7/RConn1
  Temperature Sensor7/RConn2 -- T_1.4_BRAID_START/LConn1
  Thermal Reference8/LConn1 -- Temperature Sensor8/RConn1
  Temperature Sensor8/RConn2 -- T_1.4_BRAID_END/LConn1
  Temperature Sensor10/RConn2 -- STAGE_ROTARY/LConn1
  Thermal Reference10/LConn1 -- Temperature Sensor10/RConn1
  3.1_SMARACT_STAGE_ROTARY/RConn1 -- Temperature Sensor10/LConn1
  1.6_SAMPLE_RECEIVER/RConn4 -- Heat Flow Rate Sensor87/RConn2
  Heat Flow Rate Sensor32/LConn1 -- B4/LConn1
  Temperature Sensor5/RConn2 -- T_1.3_BUSBAR/LConn1
  1.3_BUS_BAR/LConn2 -- Temperature Sensor5/LConn1
  Thermal Reference5/LConn1 -- Temperature Sensor5/RConn1
  Temperature Sensor7/LConn1 -- 1.4_BRAID_ASSEMBLY/LConn2
  Temperature Sensor8/LConn1 -- 1.4_BRAID_ASSEMBLY/LConn6
  B23/LConn1 -- Temperature Source4/LConn1
  A19/RConn1 -- Temperature Source8/LConn1
  Heat Flow Rate Sensor21/RConn2 -- A1/RConn1
  2.6_RIGID_SHIELD/RConn2 -- Heat Flow Rate Sensor43/RConn2
  B22/RConn1 -- 3.1_SMARACT_STAGE_ROTARY/LConn1
  Temperature Sensor14/RConn2 -- T_A1/LConn1
  A1/LConn1 -- Subsystem/RConn1 -- Temperature Sensor14/LConn1
  Thermal Reference14/LConn1 -- Temperature Sensor14/RConn1
  Simulink-PS Converter2/RConn1 -- A1/LConn2
  A5/LConn1 -- 1.3_BUS_BAR/RConn1 -- Temperature Sensor23/LConn1
  Temperature Sensor23/RConn2 -- T_A5/LConn1
  Thermal Reference23/LConn1 -- Temperature Sensor23/RConn1
  Simulink-PS Converter3/RConn1 -- A5/LConn2
  Heat Flow Rate Sensor22/RConn2 -- A5/RConn1
  Simulink-PS Converter4/RConn1 -- A8/LConn2
  A8/LConn1 -- Temperature Sensor24/LConn1 -- 1.4_BRAID_ASSEMBLY/RConn1
  Thermal Reference24/LConn1 -- Temperature Sensor24/RConn1
  Temperature Sensor24/RConn2 -- T_A8/LConn1
  Heat Flow Rate Sensor23/RConn2 -- A8/RConn1
  1.6_SAMPLE_RECEIVER/RConn1 -- A10/LConn1 -- Temperature Sensor32/LConn1
  Simulink-PS Converter12/RConn1 -- A10/LConn2
  Temperature Sensor32/RConn2 -- T_A10/LConn1
  Thermal Reference32/LConn1 -- Temperature Sensor32/RConn1
  Temperature Source10/LConn1 -- B4/RConn1
  1.5_PULLEY/RConn1 -- A9/LConn1 -- Temperature Sensor16/LConn1
  Simulink-PS Converter13/RConn1 -- A9/LConn2
  Temperature Sensor16/RConn2 -- T_A9/LConn1
  Heat Flow Rate Sensor24/RConn2 -- A9/RConn1
  Thermal Reference16/LConn1 -- Temperature Sensor16/RConn1
  Heat Flow Rate Sensor32/RConn2 -- 1.7_SAMPLE_HOLDER/RConn2
  Heat Flow Rate Sensor48/LConn1 -- B23/RConn1
  Heat Flow Rate Sensor48/RConn2 -- 2.6_RIGID_SHIELD/RConn6
  Heat Flow Rate Sensor31/RConn1 -- L_A11/LConn1
  Heat Flow Rate Sensor87/LConn1 -- B3/LConn1
  Heat Flow Rate Sensor48/RConn1 -- L_B23/LConn1
  Heat Flow Rate Sensor22/LConn1 -- 1.4_BRAID_ASSEMBLY/LConn1
  1.5_PULLEY/LConn1 -- Heat Flow Rate Sensor23/LConn1
  Heat Flow Rate Sensor30/LConn1 -- 1.7_SAMPLE_HOLDER/LConn1
  A11/RConn1 -- Heat Flow Rate Sensor31/RConn2
  Heat Flow Rate Sensor31/LConn1 -- 1.8_SAMPLE/LConn1 -- Solver Configuration/RConn1
  Heat Flow Rate Sensor44/RConn2 -- 4.4_INSULATOR/RConn1
  Heat Flow Rate Sensor44/LConn1 -- A18/LConn1
  Heat Flow Rate Sensor42/RConn2 -- 3.1_SMARACT_STAGE_ROTARY/RConn2
  Heat Flow Rate Sensor42/LConn1 -- A19/LConn1
  Heat Flow Rate Sensor43/LConn1 -- B22/LConn1
  Heat Flow Rate Sensor22/RConn1 -- L_A5/LConn1
  Heat Flow Rate Sensor21/RConn1 -- L_A1/LConn1
  L_A6/LConn1 -- 1.4_BRAID_ASSEMBLY/LConn3
  L_A7/LConn1 -- 1.4_BRAID_ASSEMBLY/LConn5
  L_A8/LConn1 -- Heat Flow Rate Sensor23/RConn1
  L_A9/LConn1 -- Heat Flow Rate Sensor24/RConn1
  Heat Flow Rate Sensor30/RConn1 -- L_A10/LConn1
  L_A18/LConn1 -- Heat Flow Rate Sensor44/RConn1
  Heat Flow Rate Sensor42/RConn1 -- L_A19/LConn1
  L_B3/LConn1 -- Heat Flow Rate Sensor87/RConn1
  Heat Flow Rate Sensor32/RConn1 -- L_B4/LConn1
  Heat Flow Rate Sensor43/RConn1 -- L_B22/LConn1
  Simulink-PS Converter/RConn1 -- SAMPLE_CONN/LConn2
  Thermal Reference17/LConn1 -- Temperature Sensor17/RConn1
  Temperature Sensor17/RConn2 -- T_1.5_PULLEY/LConn1
  1.5_PULLEY/LConn5 -- Temperature Sensor17/LConn1
  1.4_BRAID_ASSEMBLY/RConn3 -- B16/RConn1
  Heat Flow Rate Sensor24/LConn1 -- 1.6_SAMPLE_RECEIVER/LConn1
  A4/LConn1 -- Temperature Sensor12/LConn1 -- 1.2_BRAID_ASSEMBLY/RConn1
  Heat Flow Rate Sensor26/RConn2 -- Temperature Source/LConn1 -- A4/RConn1
  Simulink-PS Converter11/RConn1 -- A4/LConn2
  Temperature Sensor12/RConn2 -- T_A4/LConn1
  Thermal Reference12/LConn1 -- Temperature Sensor12/RConn1
  Heat Flow Rate Sensor26/RConn1 -- L_A4/LConn1
  Heat Flow Rate Sensor26/LConn1 -- 1.3_BUS_BAR/LConn1
  Heat Flow Rate Sensor21/LConn1 -- 1.2_BRAID_ASSEMBLY/LConn1
  Temperature Sensor13/RConn2 -- T_1.2_BRAID_END/LConn1
  Thermal Reference13/LConn1 -- Temperature Sensor13/RConn1
  Temperature Sensor13/LConn1 -- 1.2_BRAID_ASSEMBLY/LConn6
  Heat Flow Rate Sensor7/LConn1 -- 2.6_RIGID_SHIELD/LConn2
  Heat Flow Rate Sensor7/RConn1 -- L_B16/LConn1
  B16/LConn1 -- Heat Flow Rate Sensor7/RConn2
  A28/LConn1 -- Temperature Sensor19/LConn1 -- 2.5_BRAID_ASSEMBLY/RConn1
  Simulink-PS Converter7/RConn1 -- A28/LConn2
  Heat Flow Rate Sensor8/LConn1 -- 2.6_RIGID_SHIELD/LConn1
  Temperature Sensor19/RConn2 -- T_A28/LConn1
  Thermal Reference19/LConn1 -- Temperature Sensor19/RConn1
  Heat Flow Rate Sensor8/RConn2 -- A28/RConn1
  L_A28/LConn1 -- Heat Flow Rate Sensor8/RConn1
  A25/LConn1 -- Temperature Sensor20/LConn1 -- 2.4_RIGID_SHIELD/RConn6
  Thermal Reference20/LConn1 -- Temperature Sensor20/RConn1
  L_A25/LConn1 -- Heat Flow Rate Sensor9/RConn1
  Simulink-PS Converter8/RConn1 -- A25/LConn2
  Temperature Sensor20/RConn2 -- T_A25/LConn1
  Heat Flow Rate Sensor9/RConn2 -- A25/RConn1
  Heat Flow Rate Sensor9/LConn1 -- 2.5_BRAID_ASSEMBLY/LConn1
  A24/LConn1 -- 2.3_BRAID_ASSEMBLY/RConn1 -- Temperature Sensor21/LConn1
  Heat Flow Rate Sensor10/RConn2 -- A24/RConn1
  L_A24/LConn1 -- Heat Flow Rate Sensor10/RConn1
  Thermal Reference21/LConn1 -- Temperature Sensor21/RConn1
  Heat Flow Rate Sensor10/LConn1 -- 2.4_RIGID_SHIELD/LConn5
  Temperature Sensor21/RConn2 -- T_A24/LConn1
  Simulink-PS Converter14/RConn1 -- A24/LConn2
  A33/LConn1 -- Heat Flow Rate Sensor11/RConn2
  Heat Flow Rate Sensor11/RConn1 -- L_A33/LConn1
  A33/RConn1 -- 2.4_RIGID_SHIELD/RConn7
  Heat Flow Rate Sensor12/RConn1 -- L_B19/LConn1
  Heat Flow Rate Sensor12/LConn1 -- B19/RConn1
  B19/LConn1 -- Temperature Source3/LConn1
  Heat Flow Rate Sensor13/RConn1 -- L_B20/LConn1
  Heat Flow Rate Sensor13/LConn1 -- B20/RConn1
  B20/LConn1 -- Temperature Source5/LConn1
  Heat Flow Rate Sensor14/RConn2 -- 2.4_RIGID_SHIELD/RConn10
  Heat Flow Rate Sensor14/RConn1 -- L_B2/LConn1
  Heat Flow Rate Sensor14/LConn1 -- B2/RConn1
  B2/LConn1 -- Temperature Source6/LConn1
  2.4_RIGID_SHIELD/RConn9 -- Heat Flow Rate Sensor13/RConn2
  Heat Flow Rate Sensor12/RConn2 -- 2.4_RIGID_SHIELD/RConn8
  Heat Flow Rate Sensor15/RConn1 -- L_A32/LConn1
  Heat Flow Rate Sensor15/LConn1 -- 2.4_RIGID_SHIELD/LConn1
  A32/LConn1 -- Heat Flow Rate Sensor15/RConn2
  A32/RConn1 -- 4.2_INSULATOR/RConn1
  Heat Flow Rate Sensor16/RConn1 -- L_A31/LConn1
  Heat Flow Rate Sensor16/LConn1 -- 4.2_INSULATOR/LConn1
  A31/LConn1 -- Heat Flow Rate Sensor16/RConn2
  A31/RConn1 -- 1.3_BUS_BAR/RConn4
  Heat Flow Rate Sensor17/RConn2 -- 1.3_BUS_BAR/RConn2
  Heat Flow Rate Sensor17/RConn1 -- L_B13/LConn1
  Heat Flow Rate Sensor17/LConn1 -- B13/RConn1
  B13/LConn1 -- 2.4_RIGID_SHIELD/LConn2
  Heat Flow Rate Sensor18/RConn1 -- L_B15/LConn1
  Heat Flow Rate Sensor18/LConn1 -- B15/RConn1
  B15/LConn1 -- 2.4_RIGID_SHIELD/RConn2
  1.4_BRAID_ASSEMBLY/RConn2 -- Heat Flow Rate Sensor18/RConn2
  Heat Flow Rate Sensor19/RConn2 -- 1.3_BUS_BAR/RConn3
  Heat Flow Rate Sensor19/RConn1 -- L_B14/LConn1
  B14/LConn1 -- 2.4_RIGID_SHIELD/LConn3
  Heat Flow Rate Sensor19/LConn1 -- B14/RConn1
  A21/LConn1 -- 2.2_RIGID_SHIELD/RConn1 -- Temperature Sensor22/LConn1
  Heat Flow Rate Sensor27/RConn2 -- A21/RConn1
  L_A21/LConn1 -- Heat Flow Rate Sensor27/RConn1
  Thermal Reference22/LConn1 -- Temperature Sensor22/RConn1
  Simulink-PS Converter15/RConn1 -- A21/LConn2
  Heat Flow Rate Sensor27/LConn1 -- 2.3_BRAID_ASSEMBLY/LConn2
  Temperature Sensor22/RConn2 -- T_A21/LConn1
  A20/LConn1 -- Temperature Sensor25/LConn1 -- Subsystem/RConn2
  Simulink-PS Converter16/RConn1 -- A20/LConn2
  L_A20/LConn1 -- Heat Flow Rate Sensor28/RConn1
  Temperature Sensor25/RConn2 -- T_A20/LConn1
  Thermal Reference25/LConn1 -- Temperature Sensor25/RConn1
  Heat Flow Rate Sensor28/RConn2 -- A20/RConn1
  Heat Flow Rate Sensor29/RConn1 -- L_B18/LConn1
  B18/LConn1 -- Temperature Source7/LConn1
  Heat Flow Rate Sensor29/LConn1 -- B18/RConn1
  Heat Flow Rate Sensor29/RConn2 -- 2.3_BRAID_ASSEMBLY/RConn3
  Heat Flow Rate Sensor34/RConn1 -- L_B17/LConn1
  B17/LConn1 -- Temperature Source11/LConn1
  Heat Flow Rate Sensor34/LConn1 -- B17/RConn1
  Heat Flow Rate Sensor34/RConn2 -- 2.2_RIGID_SHIELD/RConn2
  Heat Flow Rate Sensor45/RConn2 -- 2.6_RIGID_SHIELD/RConn1
  L_A17/LConn1 -- Heat Flow Rate Sensor45/RConn1
  Heat Flow Rate Sensor45/LConn1 -- A17/LConn1
  A17/RConn1 -- 4.4_INSULATOR/LConn1
  B1/LConn1 -- 2.4_RIGID_SHIELD/LConn4
  Heat Flow Rate Sensor47/RConn1 -- L_B1/LConn1
  Heat Flow Rate Sensor47/LConn1 -- B1/RConn1
  Heat Flow Rate Sensor47/RConn2 -- 1.2_BRAID_ASSEMBLY/RConn3
  L_A2/LConn1 -- 1.2_BRAID_ASSEMBLY/LConn3
  L_A3/LConn1 -- 1.2_BRAID_ASSEMBLY/LConn5
  Temperature Source2/LConn1 -- Heat Flow Rate Sensor50/LConn1
  A34/LConn1 -- Heat Flow Rate Sensor50/RConn2
  Heat Flow Rate Sensor50/RConn1 -- L_A34/LConn1
  A34/RConn1 -- 4.3_INSULATOR/RConn1
  4.3_INSULATOR/LConn1 -- Heat Flow Rate Sensor11/LConn1
  Heat Flow Rate Sensor51/RConn1 -- L_B21/LConn1
  B21/LConn1 -- Temperature Source12/LConn1
  Heat Flow Rate Sensor51/LConn1 -- B21/RConn1
  2.5_BRAID_ASSEMBLY/RConn3 -- Heat Flow Rate Sensor51/RConn2
  Thermal Reference26/LConn1 -- Temperature Sensor26/RConn1
  Temperature Sensor26/RConn2 -- T_1.2_BRAID_START/LConn1
  Temperature Sensor26/LConn1 -- 1.2_BRAID_ASSEMBLY/LConn2
  T_COLD_HEAD/LConn1 -- Subsystem/RConn3
  Subsystem/RConn4 -- W_COLD_HEAD/LConn1
  2.3_BRAID_ASSEMBLY/LConn1 -- Heat Flow Rate Sensor28/LConn1
  Temperature Sensor27/LConn1 -- 2.2_RIGID_SHIELD/RConn3
  Temperature Sensor27/RConn2 -- T_2.2_SHIELD/LConn1
  Thermal Reference27/LConn1 -- Temperature Sensor27/RConn1
  Temperature Sensor28/RConn2 -- T_2.3.1_BRAID/LConn1
  Temperature Sensor28/LConn1 -- 2.3_BRAID_ASSEMBLY/RConn2
  Thermal Reference28/LConn1 -- Temperature Sensor28/RConn1
  Temperature Sensor29/RConn2 -- T_2.3.3_BRAID/LConn1
  2.3_BRAID_ASSEMBLY/RConn4 -- Temperature Sensor29/LConn1
  Thermal Reference29/LConn1 -- Temperature Sensor29/RConn1
  Temperature Sensor30/RConn2 -- T_2.4.3_SHIELD/LConn1
  Temperature Sensor30/LConn1 -- 2.4_RIGID_SHIELD/RConn5
  Thermal Reference30/LConn1 -- Temperature Sensor30/RConn1
  Temperature Sensor31/LConn1 -- 2.4_RIGID_SHIELD/RConn4
  Thermal Reference31/LConn1 -- Temperature Sensor31/RConn1
  Temperature Sensor31/RConn2 -- T_2.4.2_SHIELD/LConn1
  Temperature Sensor33/LConn1 -- 2.4_RIGID_SHIELD/RConn3
  Thermal Reference33/LConn1 -- Temperature Sensor33/RConn1
  Temperature Sensor33/RConn2 -- T_2.4.1_SHIELD/LConn1
  Temperature Sensor34/LConn1 -- 2.5_BRAID_ASSEMBLY/RConn2
  Thermal Reference34/LConn1 -- Temperature Sensor34/RConn1
  Temperature Sensor34/RConn2 -- T_2.5.1_BRAID/LConn1
  Temperature Sensor35/LConn1 -- 2.5_BRAID_ASSEMBLY/RConn4
  Thermal Reference35/LConn1 -- Temperature Sensor35/RConn1
  Temperature Sensor35/RConn2 -- T_2.5.3_BRAID/LConn1
  Thermal Reference36/LConn1 -- Temperature Sensor36/RConn1
  Temperature Sensor36/LConn1 -- 2.6_RIGID_SHIELD/RConn7
  Temperature Sensor36/RConn2 -- T_2.6_SHIELD/LConn1
  T_HOT_HEAD/LConn1 -- Subsystem/RConn5
  W_HOT_HEAD/LConn1 -- Subsystem/RConn6
  HEATER_4/RConn1 -- 1.4_BRAID_ASSEMBLY/LConn4
  HEATER_5/RConn1 -- 1.3_BUS_BAR/LConn3
  HEATER_6/RConn1 -- 1.2_BRAID_ASSEMBLY/LConn4
  HEATER_7/RConn1 -- 2.3_BRAID_ASSEMBLY/LConn4
  HEATER_8/RConn1 -- 2.4_RIGID_SHIELD/RConn1
  B5/RConn1 -- Temperature Source9/LConn1
  L_B5/LConn1 -- Heat Flow Rate Sensor1/RConn1
  Heat Flow Rate Sensor1/RConn2 -- 1.5_PULLEY/LConn3
  Heat Flow Rate Sensor1/LConn1 -- B5/LConn1
  L_B10.1/LConn1 -- Heat Flow Rate Sensor2/RConn1
  Heat Flow Rate Sensor2/RConn2 -- 4.7_TI_FLEXURE/LConn2
  Heat Flow Rate Sensor2/LConn1 -- B10.1/LConn1
  B10.1/RConn1 -- 1.5_PULLEY/RConn3
  B10.2/RConn1 -- 1.5_PULLEY/RConn4
  Heat Flow Rate Sensor3/RConn2 -- 4.7_TI_FLEXURE/LConn3
  L_B10.2/LConn1 -- Heat Flow Rate Sensor3/RConn1
  Heat Flow Rate Sensor3/LConn1 -- B10.2/LConn1
  B10.3/RConn1 -- 1.5_PULLEY/RConn5
  Heat Flow Rate Sensor4/RConn2 -- 4.7_TI_FLEXURE/LConn4
  L_B10.3/LConn1 -- Heat Flow Rate Sensor4/RConn1
  Heat Flow Rate Sensor4/LConn1 -- B10.3/LConn1
  Temperature Sensor3/LConn1 -- 4.7_TI_FLEXURE/LConn5 -- A37.1/LConn1
  Heat Flow Rate Sensor5/RConn2 -- A37.1/RConn1
  L_A37.1/LConn1 -- Heat Flow Rate Sensor5/RConn1
  Thermal Reference3/LConn1 -- Temperature Sensor3/RConn1
  Temperature Sensor3/RConn2 -- T_A37.1/LConn1
  Simulink-PS Converter1/RConn1 -- A37.1/LConn2
  1.5_PULLEY/RConn6 -- Heat Flow Rate Sensor5/LConn1
  Temperature Sensor4/LConn1 -- A37.2/LConn1 -- 4.7_TI_FLEXURE/LConn6
  L_A37.2/LConn1 -- Heat Flow Rate Sensor6/RConn1
  Simulink-PS Converter5/RConn1 -- A37.2/LConn2
  Temperature Sensor4/RConn2 -- T_A37.2/LConn1
  Thermal Reference4/LConn1 -- Temperature Sensor4/RConn1
  Heat Flow Rate Sensor6/RConn2 -- A37.2/RConn1
  Heat Flow Rate Sensor6/LConn1 -- 1.5_PULLEY/RConn7
  Temperature Sensor9/LConn1 -- A37.3/LConn1 -- 4.7_TI_FLEXURE/LConn7
  L_A37.3/LConn1 -- Heat Flow Rate Sensor20/RConn1
  Simulink-PS Converter6/RConn1 -- A37.3/LConn2
  Temperature Sensor9/RConn2 -- T_A37.3/LConn1
  Thermal Reference9/LConn1 -- Temperature Sensor9/RConn1
  Heat Flow Rate Sensor20/RConn2 -- A37.3/RConn1
  Heat Flow Rate Sensor20/LConn1 -- 1.5_PULLEY/RConn8
  HEATER_2/RConn1 -- 4.7_TI_FLEXURE/LConn1
  L_B9/LConn1 -- Heat Flow Rate Sensor33/RConn1
  B9/RConn1 -- Temperature Source13/LConn1
  Heat Flow Rate Sensor33/RConn2 -- 7.4 SAMPLE PCB/RConn1
  Heat Flow Rate Sensor33/LConn1 -- B9/LConn1
  L_B7/LConn1 -- Heat Flow Rate Sensor35/RConn1
  Heat Flow Rate Sensor35/LConn1 -- B7/LConn1
  Heat Flow Rate Sensor35/RConn2 -- 1.5_PULLEY/RConn2
  B7/RConn1 -- 7.1 CABLE ASSEMBLY/LConn1
  L_B8/LConn1 -- Heat Flow Rate Sensor36/RConn1
  Heat Flow Rate Sensor36/RConn2 -- 1.6_SAMPLE_RECEIVER/RConn2
  Heat Flow Rate Sensor36/LConn1 -- B8/LConn1
  B8/RConn1 -- 7.1 CABLE ASSEMBLY/LConn2
  L_A16/LConn1 -- Heat Flow Rate Sensor37/RConn1
  Heat Flow Rate Sensor37/LConn1 -- A16/LConn1
  Heat Flow Rate Sensor37/RConn2 -- 1.6_SAMPLE_RECEIVER/RConn3
  A16/RConn1 -- 7.1 CABLE ASSEMBLY/LConn3
  A15/LConn1 -- 7.1 CABLE ASSEMBLY/RConn1 -- Temperature Sensor11/LConn1
  Temperature Sensor11/RConn2 -- T_A15/LConn1
  Simulink-PS Converter9/RConn1 -- A15/LConn2
  Thermal Reference11/LConn1 -- Temperature Sensor11/RConn1
  Heat Flow Rate Sensor38/RConn1 -- L_A15/LConn1
  Heat Flow Rate Sensor38/RConn2 -- A15/RConn1
  7.3 PCB PINS/LConn1 -- Heat Flow Rate Sensor38/LConn1
  Temperature Sensor15/LConn1 -- A14/LConn1 -- 7.3 PCB PINS/RConn1
  Temperature Sensor15/RConn2 -- T_A14/LConn1
  Simulink-PS Converter10/RConn1 -- A14/LConn2
  Thermal Reference15/LConn1 -- Temperature Sensor15/RConn1
  Heat Flow Rate Sensor39/RConn1 -- L_A14/LConn1
  Heat Flow Rate Sensor39/RConn2 -- A14/RConn1
  Heat Flow Rate Sensor39/LConn1 -- 7.4 SAMPLE PCB/RConn2
  L_A13/LConn1 -- Heat Flow Rate Sensor40/RConn1
  Heat Flow Rate Sensor40/RConn2 -- 1.7_SAMPLE_HOLDER/RConn3
  Heat Flow Rate Sensor40/LConn1 -- A13/LConn1
  A13/RConn1 -- 7.4 SAMPLE PCB/LConn1
  Temperature Sensor18/LConn1 -- 7.4 SAMPLE PCB/LConn2 -- A12/LConn1
  Simulink-PS Converter17/RConn1 -- A12/LConn2
  Heat Flow Rate Sensor41/LConn1 -- 1.8_SAMPLE/RConn1
  Thermal Reference18/LConn1 -- Temperature Sensor18/RConn1
  Temperature Sensor18/RConn2 -- T_A12/LConn1
  Heat Flow Rate Sensor41/RConn2 -- A12/RConn1
  Heat Flow Rate Sensor41/RConn1 -- L_A12/LConn1
  A36/RConn1 -- 2.6_RIGID_SHIELD/LConn4
  L_A36/LConn1 -- Heat Flow Rate Sensor46/RConn1
  Heat Flow Rate Sensor46/RConn2 -- 7.1 CABLE ASSEMBLY/RConn2
  A36/LConn1 -- Heat Flow Rate Sensor46/LConn1
  Heat Flow Rate Sensor49/LConn1 -- B25/LConn1
  Heat Flow Rate Sensor49/RConn2 -- 2.6_RIGID_SHIELD/LConn3
